simulink model "mf14_100"  (R2023b)
settings: Solver=ode45  StartTime=0.0  StopTime=60  RelTol=1e-4  AbsTol=1e-6
PreLoadFcn:
  | dqesl_f14dat
undefined symbols (not defined in the file): a, b, g, Ka, Kf, Ki, Kq, Md, Mq, Mw, Swg, Ta, Tal, Ts, Uo, Vto, W1, W2, Zd, Zw
libraries: simulink3 x100
(part 1 of 10)
settings Model: Creator=The MathWorks Inc.  LastModifiedBy=dganesan
settings SolverCC: AutoScaleAbsTol=off  AlgebraicLoopSolver=TrustRegion  MaxZcPerStep=1
settings DataIOCC: ExternalInput=[]  InitialState=[]  SaveFormat=Array  SignalLoggingSaveFormat=ModelDataLogs  SaveOutput=off  SaveTime=off  ReturnWorkspaceOutputs=off
settings OptimizationCC: BlockReduction=off  BooleanDataType=off  ExpressionDepthLimit=2147483647  InitFltsAndDblsToZero=on  LifeSpan=inf
settings DebuggingCC: SaveWithParameterizedLinksMsg=none  UnderspecifiedInitializationDetection=Classic  MergeDetectMultiDrivingBlocksExec=none  SignalResolutionControl=TryResolveAllWithWarning  MultiTaskDSMMsg=warning  MultiTaskCondExecSysMsg=none  IntegerOverflowMsg=none  FcnCallInpInsideContextMsg=warning  UnconnectedInputMsg=warning  UnconnectedOutputMsg=warning  UnconnectedLineMsg=warning  StateNameClashWarn=warning  SFUnexpectedBacktrackingDiag=warning  SFNoUnconditionalDefaultTransitionDiag=warning  SFExecutionAtInitializationDiag=none  IntegerSaturationMsg=none  ArithmeticOperatorsInVariantConditions=warning
settings HardwareCC: ProdBitPerPointer=32  ProdBitPerSizeT=32  ProdBitPerPtrDiffT=32  ProdLargestAtomicFloat=None  ProdIntDivRoundTo=Undefined  ProdEndianess=Unspecified  ProdWordSize=32  ProdHWDeviceType=32-bit Generic
settings ModelReferenceCC: EnableRefExpFcnMdlSchedulingChecks=on  PropagateSignalLabelsOutOfModel=off
settings SFSimCC: SimUseLocalCustomCode=off  CustomCodeUndefinedFunction=UseInterfaceOnly
settings RTWCC: RTWUseLocalCustomCode=off  DLArmComputeVersion=19.05
settings CodeAppCC: StateflowObjectComments=on
settings GRTTargetCC: TargetFcnLib=ansi_tfl_tmw.mat  TargetLangStandard=C89/C90 (ANSI)  CombineOutputUpdateFcns=off  GRTInterface=on
settings ConfigComp: CovMetricSettings=dw  CovSaveCumulativeToWorkspaceVar=on  CovSaveSingleToWorkspaceVar=on  CovExternalEMLEnable=off

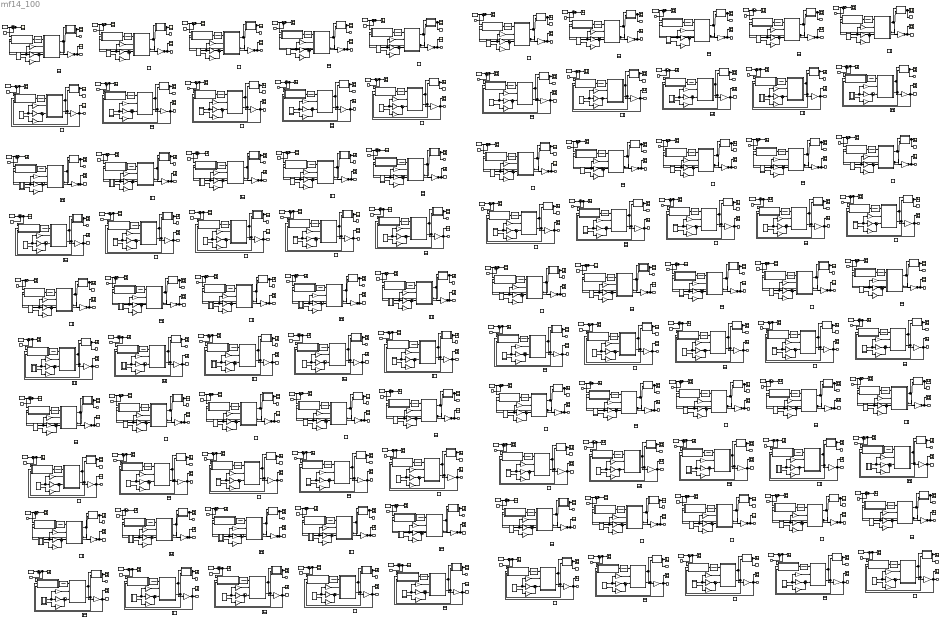
== system mf14_100 ==
  note: F-14 Flight Control
      | (an updated version of this demo is available
      | by running 'sldemo_f14')
  note: Copyright 1990-2010 The MathWorks, Inc.
  note: Copyright 1990-2010 The MathWorks, Inc.
  note: F-14 Flight Control
      | (an updated version of this demo is available
      | by running 'sldemo_f14')
  note: Copyright 1990-2010 The MathWorks, Inc.
  note: F-14 Flight Control
      | (an updated version of this demo is available
      | by running 'sldemo_f14')
  note: Copyright 1990-2010 The MathWorks, Inc.
  note: Copyright 1990-2010 The MathWorks, Inc.
  note: F-14 Flight Control
      | (an updated version of this demo is available
      | by running 'sldemo_f14')
  note: F-14 Flight Control
      | (an updated version of this demo is available
      | by running 'sldemo_f14')
  note: F-14 Flight Control
      | (an updated version of this demo is available
      | by running 'sldemo_f14')
  note: Copyright 1990-2010 The MathWorks, Inc.
  note: Copyright 1990-2010 The MathWorks, Inc.
  note: F-14 Flight Control
      | (an updated version of this demo is available
      | by running 'sldemo_f14')
  note: Copyright 1990-2010 The MathWorks, Inc.
  note: F-14 Flight Control
      | (an updated version of this demo is available
      | by running 'sldemo_f14')
  note: Copyright 1990-2010 The MathWorks, Inc.
  note: F-14 Flight Control
      | (an updated version of this demo is available
      | by running 'sldemo_f14')
  note: Copyright 1990-2010 The MathWorks, Inc.
  note: F-14 Flight Control
      | (an updated version of this demo is available
      | by running 'sldemo_f14')
  note: F-14 Flight Control
      | (an updated version of this demo is available
      | by running 'sldemo_f14')
  note: F-14 Flight Control
      | (an updated version of this demo is available
      | by running 'sldemo_f14')
  note: F-14 Flight Control
      | (an updated version of this demo is available
      | by running 'sldemo_f14')
  note: Copyright 1990-2010 The MathWorks, Inc.
  note: Copyright 1990-2010 The MathWorks, Inc.
  note: F-14 Flight Control
      | (an updated version of this demo is available
      | by running 'sldemo_f14')
  note: Copyright 1990-2010 The MathWorks, Inc.
  note: Copyright 1990-2010 The MathWorks, Inc.
  note: F-14 Flight Control
      | (an updated version of this demo is available
      | by running 'sldemo_f14')
  note: Copyright 1990-2010 The MathWorks, Inc.
  note: F-14 Flight Control
      | (an updated version of this demo is available
      | by running 'sldemo_f14')
  note: Copyright 1990-2010 The MathWorks, Inc.
  note: Copyright 1990-2010 The MathWorks, Inc.
  note: F-14 Flight Control
      | (an updated version of this demo is available
      | by running 'sldemo_f14')
  note: Copyright 1990-2010 The MathWorks, Inc.
  note: F-14 Flight Control
      | (an updated version of this demo is available
      | by running 'sldemo_f14')
  note: Copyright 1990-2010 The MathWorks, Inc.
  note: F-14 Flight Control
      | (an updated version of this demo is available
      | by running 'sldemo_f14')
  note: Copyright 1990-2010 The MathWorks, Inc.
  note: F-14 Flight Control
      | (an updated version of this demo is available
      | by running 'sldemo_f14')
  note: F-14 Flight Control
      | (an updated version of this demo is available
      | by running 'sldemo_f14')
  note: F-14 Flight Control
      | (an updated version of this demo is available
      | by running 'sldemo_f14')
  note: F-14 Flight Control
      | (an updated version of this demo is available
      | by running 'sldemo_f14')
  note: Copyright 1990-2010 The MathWorks, Inc.
  note: Copyright 1990-2010 The MathWorks, Inc.
  note: F-14 Flight Control
      | (an updated version of this demo is available
      | by running 'sldemo_f14')
  note: Copyright 1990-2010 The MathWorks, Inc.
  note: Copyright 1990-2010 The MathWorks, Inc.
  note: F-14 Flight Control
      | (an updated version of this demo is available
      | by running 'sldemo_f14')
  note: Copyright 1990-2010 The MathWorks, Inc.
  note: F-14 Flight Control
      | (an updated version of this demo is available
      | by running 'sldemo_f14')
  note: Copyright 1990-2010 The MathWorks, Inc.
  note: Copyright 1990-2010 The MathWorks, Inc.
  note: F-14 Flight Control
      | (an updated version of this demo is available
      | by running 'sldemo_f14')
  note: Copyright 1990-2010 The MathWorks, Inc.
  note: F-14 Flight Control
      | (an updated version of this demo is available
      | by running 'sldemo_f14')
  note: Copyright 1990-2010 The MathWorks, Inc.
  note: F-14 Flight Control
      | (an updated version of this demo is available
      | by running 'sldemo_f14')
  note: Copyright 1990-2010 The MathWorks, Inc.
  note: F-14 Flight Control
      | (an updated version of this demo is available
      | by running 'sldemo_f14')
  note: F-14 Flight Control
      | (an updated version of this demo is available
      | by running 'sldemo_f14')
  note: F-14 Flight Control
      | (an updated version of this demo is available
      | by running 'sldemo_f14')
  note: F-14 Flight Control
      | (an updated version of this demo is available
      | by running 'sldemo_f14')
  note: Copyright 1990-2010 The MathWorks, Inc.
  note: Copyright 1990-2010 The MathWorks, Inc.
  note: F-14 Flight Control
      | (an updated version of this demo is available
      | by running 'sldemo_f14')
  note: Copyright 1990-2010 The MathWorks, Inc.
  note: Copyright 1990-2010 The MathWorks, Inc.
  note: F-14 Flight Control
      | (an updated version of this demo is available
      | by running 'sldemo_f14')
  note: Copyright 1990-2010 The MathWorks, Inc.
  note: F-14 Flight Control
      | (an updated version of this demo is available
      | by running 'sldemo_f14')
  note: Copyright 1990-2010 The MathWorks, Inc.
  note: Copyright 1990-2010 The MathWorks, Inc.
  note: F-14 Flight Control
      | (an updated version of this demo is available
      | by running 'sldemo_f14')
  note: Copyright 1990-2010 The MathWorks, Inc.
  note: F-14 Flight Control
      | (an updated version of this demo is available
      | by running 'sldemo_f14')
  note: Copyright 1990-2010 The MathWorks, Inc.
  note: F-14 Flight Control
      | (an updated version of this demo is available
      | by running 'sldemo_f14')
  note: Copyright 1990-2010 The MathWorks, Inc.
  note: F-14 Flight Control
      | (an updated version of this demo is available
      | by running 'sldemo_f14')
  note: F-14 Flight Control
      | (an updated version of this demo is available
      | by running 'sldemo_f14')
  note: F-14 Flight Control
      | (an updated version of this demo is available
      | by running 'sldemo_f14')
  note: F-14 Flight Control
      | (an updated version of this demo is available
      | by running 'sldemo_f14')
  note: Copyright 1990-2010 The MathWorks, Inc.
  note: Copyright 1990-2010 The MathWorks, Inc.
  note: F-14 Flight Control
      | (an updated version of this demo is available
      | by running 'sldemo_f14')
  note: Copyright 1990-2010 The MathWorks, Inc.
  note: Copyright 1990-2010 The MathWorks, Inc.
  note: F-14 Flight Control
      | (an updated version of this demo is available
      | by running 'sldemo_f14')
  note: Copyright 1990-2010 The MathWorks, Inc.
  note: F-14 Flight Control
      | (an updated version of this demo is available
      | by running 'sldemo_f14')
  note: Copyright 1990-2010 The MathWorks, Inc.
  note: Copyright 1990-2010 The MathWorks, Inc.
  note: F-14 Flight Control
      | (an updated version of this demo is available
      | by running 'sldemo_f14')
  note: Copyright 1990-2010 The MathWorks, Inc.
  note: F-14 Flight Control
      | (an updated version of this demo is available
      | by running 'sldemo_f14')
  note: Copyright 1990-2010 The MathWorks, Inc.
  note: F-14 Flight Control
      | (an updated version of this demo is available
      | by running 'sldemo_f14')
  note: Copyright 1990-2010 The MathWorks, Inc.
  note: F-14 Flight Control
      | (an updated version of this demo is available
      | by running 'sldemo_f14')
  note: F-14 Flight Control
      | (an updated version of this demo is available
      | by running 'sldemo_f14')
  note: Copyright 1990-2010 The MathWorks, Inc.
  note: F-14 Flight Control
      | (an updated version of this demo is available
      | by running 'sldemo_f14')
  note: F-14 Flight Control
      | (an updated version of this demo is available
      | by running 'sldemo_f14')
  note: F-14 Flight Control
      | (an updated version of this demo is available
      | by running 'sldemo_f14')
  note: Copyright 1990-2010 The MathWorks, Inc.
  note: Copyright 1990-2010 The MathWorks, Inc.
  note: Copyright 1990-2010 The MathWorks, Inc.
  note: Copyright 1990-2010 The MathWorks, Inc.
  note: Copyright 1990-2010 The MathWorks, Inc.
  note: F-14 Flight Control
      | (an updated version of this demo is available
      | by running 'sldemo_f14')
  note: Copyright 1990-2010 The MathWorks, Inc.
  note: Copyright 1990-2010 The MathWorks, Inc.
  note: F-14 Flight Control
      | (an updated version of this demo is available
      | by running 'sldemo_f14')
  note: F-14 Flight Control
      | (an updated version of this demo is available
      | by running 'sldemo_f14')
  note: F-14 Flight Control
      | (an updated version of this demo is available
      | by running 'sldemo_f14')
  note: F-14 Flight Control
      | (an updated version of this demo is available
      | by running 'sldemo_f14')
  note: F-14 Flight Control
      | (an updated version of this demo is available
      | by running 'sldemo_f14')
  note: Copyright 1990-2010 The MathWorks, Inc.
  note: Copyright 1990-2010 The MathWorks, Inc.
  note: F-14 Flight Control
      | (an updated version of this demo is available
      | by running 'sldemo_f14')
  note: Copyright 1990-2010 The MathWorks, Inc.
  note: Copyright 1990-2010 The MathWorks, Inc.
  note: F-14 Flight Control
      | (an updated version of this demo is available
      | by running 'sldemo_f14')
  note: F-14 Flight Control
      | (an updated version of this demo is available
      | by running 'sldemo_f14')
  note: Copyright 1990-2010 The MathWorks, Inc.
  note: F-14 Flight Control
      | (an updated version of this demo is available
      | by running 'sldemo_f14')
  note: Copyright 1990-2010 The MathWorks, Inc.
  note: F-14 Flight Control
      | (an updated version of this demo is available
      | by running 'sldemo_f14')
  note: F-14 Flight Control
      | (an updated version of this demo is available
      | by running 'sldemo_f14')
  note: Copyright 1990-2010 The MathWorks, Inc.
  note: F-14 Flight Control
      | (an updated version of this demo is available
      | by running 'sldemo_f14')
  note: F-14 Flight Control
      | (an updated version of this demo is available
      | by running 'sldemo_f14')
  note: F-14 Flight Control
      | (an updated version of this demo is available
      | by running 'sldemo_f14')
  note: Copyright 1990-2010 The MathWorks, Inc.
  note: Copyright 1990-2010 The MathWorks, Inc.
  note: F-14 Flight Control
      | (an updated version of this demo is available
      | by running 'sldemo_f14')
  note: F-14 Flight Control
      | (an updated version of this demo is available
      | by running 'sldemo_f14')
  note: F-14 Flight Control
      | (an updated version of this demo is available
      | by running 'sldemo_f14')
  note: F-14 Flight Control
      | (an updated version of this demo is available
      | by running 'sldemo_f14')
  note: Copyright 1990-2010 The MathWorks, Inc.
  note: F-14 Flight Control
      | (an updated version of this demo is available
      | by running 'sldemo_f14')
  note: Copyright 1990-2010 The MathWorks, Inc.
  note: Copyright 1990-2010 The MathWorks, Inc.
  note: F-14 Flight Control
      | (an updated version of this demo is available
      | by running 'sldemo_f14')
  note: Copyright 1990-2010 The MathWorks, Inc.
  note: Copyright 1990-2010 The MathWorks, Inc.
  note: Copyright 1990-2010 The MathWorks, Inc.
  note: F-14 Flight Control
      | (an updated version of this demo is available
      | by running 'sldemo_f14')
  note: Copyright 1990-2010 The MathWorks, Inc.
  note: Copyright 1990-2010 The MathWorks, Inc.
  note: Copyright 1990-2010 The MathWorks, Inc.
  note: F-14 Flight Control
      | (an updated version of this demo is available
      | by running 'sldemo_f14')
  note: F-14 Flight Control
      | (an updated version of this demo is available
      | by running 'sldemo_f14')
  note: Copyright 1990-2010 The MathWorks, Inc.
  note: F-14 Flight Control
      | (an updated version of this demo is available
      | by running 'sldemo_f14')
  note: Copyright 1990-2010 The MathWorks, Inc.
  note: Copyright 1990-2010 The MathWorks, Inc.
  note: F-14 Flight Control
      | (an updated version of this demo is available
      | by running 'sldemo_f14')
  note: Copyright 1990-2010 The MathWorks, Inc.
  note: Copyright 1990-2010 The MathWorks, Inc.
  note: Copyright 1990-2010 The MathWorks, Inc.
  note: F-14 Flight Control
      | (an updated version of this demo is available
      | by running 'sldemo_f14')
  note: F-14 Flight Control
      | (an updated version of this demo is available
      | by running 'sldemo_f14')
  note: Copyright 1990-2010 The MathWorks, Inc.
  note: Copyright 1990-2010 The MathWorks, Inc.
  note: Copyright 1990-2010 The MathWorks, Inc.
  note: F-14 Flight Control
      | (an updated version of this demo is available
      | by running 'sldemo_f14')
  note: Copyright 1990-2010 The MathWorks, Inc.
  note: F-14 Flight Control
      | (an updated version of this demo is available
      | by running 'sldemo_f14')
  note: F-14 Flight Control
      | (an updated version of this demo is available
      | by running 'sldemo_f14')
  note: Copyright 1990-2010 The MathWorks, Inc.
  note: Copyright 1990-2010 The MathWorks, Inc.
  note: Copyright 1990-2010 The MathWorks, Inc.
  note: F-14 Flight Control
      | (an updated version of this demo is available
      | by running 'sldemo_f14')
  note: Copyright 1990-2010 The MathWorks, Inc.
  note: Copyright 1990-2010 The MathWorks, Inc.
  note: F-14 Flight Control
      | (an updated version of this demo is available
      | by running 'sldemo_f14')
  note: F-14 Flight Control
      | (an updated version of this demo is available
      | by running 'sldemo_f14')
  note: F-14 Flight Control
      | (an updated version of this demo is available
      | by running 'sldemo_f14')
  note: F-14 Flight Control
      | (an updated version of this demo is available
      | by running 'sldemo_f14')
  note: F-14 Flight Control
      | (an updated version of this demo is available
      | by running 'sldemo_f14')
  note: F-14 Flight Control
      | (an updated version of this demo is available
      | by running 'sldemo_f14')
  note: Copyright 1990-2010 The MathWorks, Inc.
  note: Copyright 1990-2010 The MathWorks, Inc.
  note: Copyright 1990-2010 The MathWorks, Inc.
  note: F-14 Flight Control
      | (an updated version of this demo is available
      | by running 'sldemo_f14')
  note: Copyright 1990-2010 The MathWorks, Inc.
  note: Copyright 1990-2010 The MathWorks, Inc.
  note: F-14 Flight Control
      | (an updated version of this demo is available
      | by running 'sldemo_f14')
  note: F-14 Flight Control
      | (an updated version of this demo is available
      | by running 'sldemo_f14')
  note: F-14 Flight Control
      | (an updated version of this demo is available
      | by running 'sldemo_f14')
  note: F-14 Flight Control
      | (an updated version of this demo is available
      | by running 'sldemo_f14')
  note: Copyright 1990-2010 The MathWorks, Inc.
  note: F-14 Flight Control
      | (an updated version of this demo is available
      | by running 'sldemo_f14')
  note: F-14 Flight Control
      | (an updated version of this demo is available
      | by running 'sldemo_f14')
  note: F-14 Flight Control
      | (an updated version of this demo is available
      | by running 'sldemo_f14')
  note: Copyright 1990-2010 The MathWorks, Inc.
  note: Copyright 1990-2010 The MathWorks, Inc.
  note: Copyright 1990-2010 The MathWorks, Inc.
  u : Inport
  u1 : Inport  Port=2
  u2 : Inport  Port=3
  u3 : Inport  Port=4
  u4 : Inport  Port=5
  u5 : Inport  Port=6
  u6 : Inport  Port=7
  u7 : Inport  Port=8
  u8 : Inport  Port=9
  u9 : Inport  Port=10
  u10 : Inport  Port=11
  u11 : Inport  Port=12
  u12 : Inport  Port=13
  u13 : Inport  Port=14
  u14 : Inport  Port=15
  u15 : Inport  Port=16
  u16 : Inport  Port=17
  u17 : Inport  Port=18
  u18 : Inport  Port=19
  u19 : Inport  Port=20
  u20 : Inport  Port=21
  u21 : Inport  Port=22
  u22 : Inport  Port=23
  u23 : Inport  Port=24
  u24 : Inport  Port=25
  u25 : Inport  Port=26
  u26 : Inport  Port=27
  u27 : Inport  Port=28
  u28 : Inport  Port=29
  u29 : Inport  Port=30
  u30 : Inport  Port=31
  u31 : Inport  Port=32
  u32 : Inport  Port=33
  u33 : Inport  Port=34
  u34 : Inport  Port=35
  u35 : Inport  Port=36
  u36 : Inport  Port=37
  u37 : Inport  Port=38
  u38 : Inport  Port=39
  u39 : Inport  Port=40
  u40 : Inport  Port=41
  u41 : Inport  Port=42
  u42 : Inport  Port=43
  u43 : Inport  Port=44
  u44 : Inport  Port=45
  u45 : Inport  Port=46
  u46 : Inport  Port=47
  u47 : Inport  Port=48
  u48 : Inport  Port=49
  u49 : Inport  Port=50
  u50 : Inport  Port=51
  u51 : Inport  Port=52
  u52 : Inport  Port=53
  u53 : Inport  Port=54
  u54 : Inport  Port=55
  u55 : Inport  Port=56
  u56 : Inport  Port=57
  u57 : Inport  Port=58
  u58 : Inport  Port=59
  u59 : Inport  Port=60
  u60 : Inport  Port=61
  u61 : Inport  Port=62
  u62 : Inport  Port=63
  u63 : Inport  Port=64
  u64 : Inport  Port=65
  u65 : Inport  Port=66
  u66 : Inport  Port=67
  u67 : Inport  Port=68
  u68 : Inport  Port=69
  u69 : Inport  Port=70
  u70 : Inport  Port=71
  u71 : Inport  Port=72
  u72 : Inport  Port=73
  u73 : Inport  Port=74
  u74 : Inport  Port=75
  u75 : Inport  Port=76
  u76 : Inport  Port=77
  u77 : Inport  Port=78
  u78 : Inport  Port=79
  u79 : Inport  Port=80
  u80 : Inport  Port=81
  u81 : Inport  Port=82
  u82 : Inport  Port=83
  u83 : Inport  Port=84
  u84 : Inport  Port=85
  u85 : Inport  Port=86
  u86 : Inport  Port=87
  u87 : Inport  Port=88
  u88 : Inport  Port=89
  u89 : Inport  Port=90
  u90 : Inport  Port=91
  u91 : Inport  Port=92
  u92 : Inport  Port=93
  u93 : Inport  Port=94
  u94 : Inport  Port=95
  u95 : Inport  Port=96
  u96 : Inport  Port=97
  u97 : Inport  Port=98
  u98 : Inport  Port=99
  u99 : Inport  Port=100
  Actuator Model{,1..99} (100 alike) : TransferFcn  Denominator=[ Ta, 1]
  Aircraft Dynamics Model : Subsystem
  Aircraft Dynamics Model1 : Subsystem
  Aircraft Dynamics Model10 : Subsystem
  Aircraft Dynamics Model11 : Subsystem
  Aircraft Dynamics Model12 : Subsystem
  Aircraft Dynamics Model13 : Subsystem
  Aircraft Dynamics Model14 : Subsystem
  Aircraft Dynamics Model15 : Subsystem
  Aircraft Dynamics Model16 : Subsystem
  Aircraft Dynamics Model17 : Subsystem
  Aircraft Dynamics Model18 : Subsystem
  Aircraft Dynamics Model19 : Subsystem
  Aircraft Dynamics Model2 : Subsystem
  Aircraft Dynamics Model20 : Subsystem
  Aircraft Dynamics Model21 : Subsystem
  Aircraft Dynamics Model22 : Subsystem
  Aircraft Dynamics Model23 : Subsystem
  Aircraft Dynamics Model24 : Subsystem
  Aircraft Dynamics Model25 : Subsystem
  Aircraft Dynamics Model26 : Subsystem
  Aircraft Dynamics Model27 : Subsystem
  Aircraft Dynamics Model28 : Subsystem
  Aircraft Dynamics Model29 : Subsystem
  Aircraft Dynamics Model3 : Subsystem
  Aircraft Dynamics Model30 : Subsystem
  Aircraft Dynamics Model31 : Subsystem
  Aircraft Dynamics Model32 : Subsystem
  Aircraft Dynamics Model33 : Subsystem
  Aircraft Dynamics Model34 : Subsystem
  Aircraft Dynamics Model35 : Subsystem
  Aircraft Dynamics Model36 : Subsystem
  Aircraft Dynamics Model37 : Subsystem
  Aircraft Dynamics Model38 : Subsystem
  Aircraft Dynamics Model39 : Subsystem
  Aircraft Dynamics Model4 : Subsystem
  Aircraft Dynamics Model40 : Subsystem
  Aircraft Dynamics Model41 : Subsystem
  Aircraft Dynamics Model42 : Subsystem
  Aircraft Dynamics Model43 : Subsystem
  Aircraft Dynamics Model44 : Subsystem
  Aircraft Dynamics Model45 : Subsystem
  Aircraft Dynamics Model46 : Subsystem
  Aircraft Dynamics Model47 : Subsystem
  Aircraft Dynamics Model48 : Subsystem
  Aircraft Dynamics Model49 : Subsystem
  Aircraft Dynamics Model5 : Subsystem
  Aircraft Dynamics Model50 : Subsystem
  Aircraft Dynamics Model51 : Subsystem
  Aircraft Dynamics Model52 : Subsystem
  Aircraft Dynamics Model53 : Subsystem
  Aircraft Dynamics Model54 : Subsystem
  Aircraft Dynamics Model55 : Subsystem
  Aircraft Dynamics Model56 : Subsystem
  Aircraft Dynamics Model57 : Subsystem
  Aircraft Dynamics Model58 : Subsystem
  Aircraft Dynamics Model59 : Subsystem
  Aircraft Dynamics Model6 : Subsystem
  Aircraft Dynamics Model60 : Subsystem
  Aircraft Dynamics Model61 : Subsystem
  Aircraft Dynamics Model62 : Subsystem
  Aircraft Dynamics Model63 : Subsystem
  Aircraft Dynamics Model64 : Subsystem
  Aircraft Dynamics Model65 : Subsystem
  Aircraft Dynamics Model66 : Subsystem
  Aircraft Dynamics Model67 : Subsystem
  Aircraft Dynamics Model68 : Subsystem
  Aircraft Dynamics Model69 : Subsystem
  Aircraft Dynamics Model7 : Subsystem
  Aircraft Dynamics Model70 : Subsystem
  Aircraft Dynamics Model71 : Subsystem
  Aircraft Dynamics Model72 : Subsystem
  Aircraft Dynamics Model73 : Subsystem
  Aircraft Dynamics Model74 : Subsystem
  Aircraft Dynamics Model75 : Subsystem
  Aircraft Dynamics Model76 : Subsystem
  Aircraft Dynamics Model77 : Subsystem
  Aircraft Dynamics Model78 : Subsystem
  Aircraft Dynamics Model79 : Subsystem
  Aircraft Dynamics Model8 : Subsystem
  Aircraft Dynamics Model80 : Subsystem
  Aircraft Dynamics Model81 : Subsystem
  Aircraft Dynamics Model82 : Subsystem
  Aircraft Dynamics Model83 : Subsystem
  Aircraft Dynamics Model84 : Subsystem
  Aircraft Dynamics Model85 : Subsystem
  Aircraft Dynamics Model86 : Subsystem
  Aircraft Dynamics Model87 : Subsystem
  Aircraft Dynamics Model88 : Subsystem
  Aircraft Dynamics Model89 : Subsystem
  Aircraft Dynamics Model9 : Subsystem
  Aircraft Dynamics Model90 : Subsystem
  Aircraft Dynamics Model91 : Subsystem
  Aircraft Dynamics Model92 : Subsystem
  Aircraft Dynamics Model93 : Subsystem
  Aircraft Dynamics Model94 : Subsystem
  Aircraft Dynamics Model95 : Subsystem
  Aircraft Dynamics Model96 : Subsystem
  Aircraft Dynamics Model97 : Subsystem
  Aircraft Dynamics Model98 : Subsystem
  Aircraft Dynamics Model99 : Subsystem
  Angle of Attack{,1..99} (100 alike) : Scope
  Controller : Subsystem
  Controller1 : Subsystem
  Controller10 : Subsystem
  Controller11 : Subsystem
  Controller12 : Subsystem
  Controller13 : Subsystem
  Controller14 : Subsystem
  Controller15 : Subsystem
  Controller16 : Subsystem
  Controller17 : Subsystem
  Controller18 : Subsystem
  Controller19 : Subsystem
  Controller2 : Subsystem
  Controller20 : Subsystem
  Controller21 : Subsystem
  Controller22 : Subsystem
  Controller23 : Subsystem
  Controller24 : Subsystem
  Controller25 : Subsystem
  Controller26 : Subsystem
  Controller27 : Subsystem
  Controller28 : Subsystem
  Controller29 : Subsystem
  Controller3 : Subsystem
  Controller30 : Subsystem
  Controller31 : Subsystem
  Controller32 : Subsystem
  Controller33 : Subsystem
  Controller34 : Subsystem
  Controller35 : Subsystem
  Controller36 : Subsystem
  Controller37 : Subsystem
  Controller38 : Subsystem
  Controller39 : Subsystem
  Controller4 : Subsystem
  Controller40 : Subsystem
  Controller41 : Subsystem
  Controller42 : Subsystem
  Controller43 : Subsystem
  Controller44 : Subsystem
  Controller45 : Subsystem
  Controller46 : Subsystem
  Controller47 : Subsystem
  Controller48 : Subsystem
  Controller49 : Subsystem
  Controller5 : Subsystem
  Controller50 : Subsystem
  Controller51 : Subsystem
  Controller52 : Subsystem
  Controller53 : Subsystem
  Controller54 : Subsystem
  Controller55 : Subsystem
  Controller56 : Subsystem
  Controller57 : Subsystem
  Controller58 : Subsystem
  Controller59 : Subsystem
  Controller6 : Subsystem
  Controller60 : Subsystem
  Controller61 : Subsystem
  Controller62 : Subsystem
  Controller63 : Subsystem
  Controller64 : Subsystem
  Controller65 : Subsystem
  Controller66 : Subsystem
  Controller67 : Subsystem
  Controller68 : Subsystem
  Controller69 : Subsystem
  Controller7 : Subsystem
  Controller70 : Subsystem
  Controller71 : Subsystem
  Controller72 : Subsystem
  Controller73 : Subsystem
  Controller74 : Subsystem
  Controller75 : Subsystem
  Controller76 : Subsystem
  Controller77 : Subsystem
  Controller78 : Subsystem
  Controller79 : Subsystem
  Controller8 : Subsystem
  Controller80 : Subsystem
  Controller81 : Subsystem
  Controller82 : Subsystem
  Controller83 : Subsystem
  Controller84 : Subsystem
  Controller85 : Subsystem
  Controller86 : Subsystem
  Controller87 : Subsystem
  Controller88 : Subsystem
  Controller89 : Subsystem
  Controller9 : Subsystem
  Controller90 : Subsystem
  Controller91 : Subsystem
  Controller92 : Subsystem
  Controller93 : Subsystem
  Controller94 : Subsystem
  Controller95 : Subsystem
  Controller96 : Subsystem
  Controller97 : Subsystem
  Controller98 : Subsystem
  Controller99 : Subsystem
  Dryden Wind Gust Models : Subsystem
  Dryden Wind Gust Models1 : Subsystem
  Dryden Wind Gust Models10 : Subsystem
  Dryden Wind Gust Models11 : Subsystem
  Dryden Wind Gust Models12 : Subsystem
  Dryden Wind Gust Models13 : Subsystem
  Dryden Wind Gust Models14 : Subsystem
  Dryden Wind Gust Models15 : Subsystem
  Dryden Wind Gust Models16 : Subsystem
  Dryden Wind Gust Models17 : Subsystem
  Dryden Wind Gust Models18 : Subsystem
  Dryden Wind Gust Models19 : Subsystem
  Dryden Wind Gust Models2 : Subsystem
  Dryden Wind Gust Models20 : Subsystem
  Dryden Wind Gust Models21 : Subsystem
  Dryden Wind Gust Models22 : Subsystem
  Dryden Wind Gust Models23 : Subsystem
  Dryden Wind Gust Models24 : Subsystem
  Dryden Wind Gust Models25 : Subsystem
  Dryden Wind Gust Models26 : Subsystem
  Dryden Wind Gust Models27 : Subsystem
  Dryden Wind Gust Models28 : Subsystem
  Dryden Wind Gust Models29 : Subsystem
  Dryden Wind Gust Models3 : Subsystem
  Dryden Wind Gust Models30 : Subsystem
  Dryden Wind Gust Models31 : Subsystem
  Dryden Wind Gust Models32 : Subsystem
  Dryden Wind Gust Models33 : Subsystem
  Dryden Wind Gust Models34 : Subsystem
  Dryden Wind Gust Models35 : Subsystem
  Dryden Wind Gust Models36 : Subsystem
  Dryden Wind Gust Models37 : Subsystem
  Dryden Wind Gust Models38 : Subsystem
  Dryden Wind Gust Models39 : Subsystem
  Dryden Wind Gust Models4 : Subsystem
  Dryden Wind Gust Models40 : Subsystem
  Dryden Wind Gust Models41 : Subsystem
  Dryden Wind Gust Models42 : Subsystem
  Dryden Wind Gust Models43 : Subsystem
  Dryden Wind Gust Models44 : Subsystem
  Dryden Wind Gust Models45 : Subsystem
  Dryden Wind Gust Models46 : Subsystem
  Dryden Wind Gust Models47 : Subsystem
  Dryden Wind Gust Models48 : Subsystem
  Dryden Wind Gust Models49 : Subsystem
  Dryden Wind Gust Models5 : Subsystem
  Dryden Wind Gust Models50 : Subsystem
  Dryden Wind Gust Models51 : Subsystem
  Dryden Wind Gust Models52 : Subsystem
  Dryden Wind Gust Models53 : Subsystem
  Dryden Wind Gust Models54 : Subsystem
  Dryden Wind Gust Models55 : Subsystem
  Dryden Wind Gust Models56 : Subsystem
  Dryden Wind Gust Models57 : Subsystem
  Dryden Wind Gust Models58 : Subsystem
  Dryden Wind Gust Models59 : Subsystem
  Dryden Wind Gust Models6 : Subsystem
  Dryden Wind Gust Models60 : Subsystem
  Dryden Wind Gust Models61 : Subsystem
  Dryden Wind Gust Models62 : Subsystem
  Dryden Wind Gust Models63 : Subsystem
  Dryden Wind Gust Models64 : Subsystem
  Dryden Wind Gust Models65 : Subsystem
  Dryden Wind Gust Models66 : Subsystem
  Dryden Wind Gust Models67 : Subsystem
  Dryden Wind Gust Models68 : Subsystem
  Dryden Wind Gust Models69 : Subsystem
  Dryden Wind Gust Models7 : Subsystem
  Dryden Wind Gust Models70 : Subsystem
  Dryden Wind Gust Models71 : Subsystem
  Dryden Wind Gust Models72 : Subsystem
  Dryden Wind Gust Models73 : Subsystem
  Dryden Wind Gust Models74 : Subsystem
  Dryden Wind Gust Models75 : Subsystem
  Dryden Wind Gust Models76 : Subsystem
  Dryden Wind Gust Models77 : Subsystem
  Dryden Wind Gust Models78 : Subsystem
  Dryden Wind Gust Models79 : Subsystem
  Dryden Wind Gust Models8 : Subsystem
  Dryden Wind Gust Models80 : Subsystem
  Dryden Wind Gust Models81 : Subsystem
  Dryden Wind Gust Models82 : Subsystem
  Dryden Wind Gust Models83 : Subsystem
  Dryden Wind Gust Models84 : Subsystem
  Dryden Wind Gust Models85 : Subsystem
  Dryden Wind Gust Models86 : Subsystem
  Dryden Wind Gust Models87 : Subsystem
  Dryden Wind Gust Models88 : Subsystem
  Dryden Wind Gust Models89 : Subsystem
  Dryden Wind Gust Models9 : Subsystem
  Dryden Wind Gust Models90 : Subsystem
  Dryden Wind Gust Models91 : Subsystem
  Dryden Wind Gust Models92 : Subsystem
  Dryden Wind Gust Models93 : Subsystem
  Dryden Wind Gust Models94 : Subsystem
  Dryden Wind Gust Models95 : Subsystem
  Dryden Wind Gust Models96 : Subsystem
  Dryden Wind Gust Models97 : Subsystem
  Dryden Wind Gust Models98 : Subsystem
  Dryden Wind Gust Models99 : Subsystem
  Gain{,3,8,12,15,20,24,27,33,38,40,44,47,53,57,60,63,67,72,78,80,84,87,93,97,100,103,107,112,118,120,124,127,133,137,140,143,147,152,158,160,164,167,173,177,180,183,187,192,198,200,203,206,210,216,222,224..225,229,232,239,243,247,250,254,257,260,266,269,273,276,283,287,291,294,298,304,310,313,317,320,323,327,332,335,339,342,349,353,357,360,364,370,376,378..379,383,386,393,397} (100 alike) : Gain  Gain=Zw  SaturateOnIntegerOverflow=on  OutDataTypeStr=Inherit: Same as input  ParamDataTypeStr=Inherit: Same as input
  Gain{1,4,9,13,16,21,25,28,34,39,41,45,48,54,58,61,68,73..74,79,81,85,88,94,98,101,108,113..114,119,121,125,128,134,138,141,148,153..154,159,161,165,168,174,178,181,188,193..194,199,201,204,211,217..218,223,226,230,233,235,240,244,248,255,261..262,267..268,270,274,277,284,288,292,299,305..306,311,314,318,321,328,333..334,336,340,343,350,354,358,365,371..372,377,380,384,387,389,394,398} (100 alike) : Gain  Gain=Mq  SaturateOnIntegerOverflow=on  OutDataTypeStr=Inherit: Same as input  ParamDataTypeStr=Inherit: Same as input
  Gain{2,6,10,14,18,22,26,30,32,36,42,46,50,52,55,59,64,66,70,76,82,86,90,92,95,99,104,106,110,116,122,126,130,132,135,139,144,146,150,156,162,166,170,172,175,179,184,186,190,196,202,207,209,214,220,227,231,236,238,241,245..246,251,253,258,264,271,275,280,282,285,289..290,295,297,302,308,312,315,319,324,326,330,337,341,346,348,351,355..356,361,363,368,374,381,385,390,392,395,399} (100 alike) : Gain  Gain=Mw  SaturateOnIntegerOverflow=on  OutDataTypeStr=Inherit: Same as input  ParamDataTypeStr=Inherit: Same as input
  Gain{5,7,11,17,19,23,29,31,35,37,43,49,51,56,62,65,69,71,75,77,83,89,91,96,102,105,109,111,115,117,123,129,131,136,142,145,149,151,155,157,163,169,171,176,182,185,189,191,195,197,205,208,212..213,215,219,221,228,234,237,242,249,252,256,259,263,265,272,278..279,281,286,293,296,300..301,303,307,309,316,322,325,329,331,338,344..345,347,352,359,362,366..367,369,373,375,382,388,391,396} (100 alike) : Gain  Gain=1/Uo  SaturateOnIntegerOverflow=on  OutDataTypeStr=Inherit: Same as input  ParamDataTypeStr=Inherit: Same as input
  More Info1 : Subsystem
      settings: OpenFcn=showdemo('sldemo_f14')
      mask Display: disp('?')
  More Info10 : Subsystem
      settings: OpenFcn=showdemo('sldemo_f14')
      mask Display: disp('?')
  More Info100 : Subsystem
      settings: OpenFcn=showdemo('sldemo_f14')
      mask Display: disp('?')
  More Info11 : Subsystem
      settings: OpenFcn=showdemo('sldemo_f14')
      mask Display: disp('?')
  More Info12 : Subsystem
      settings: OpenFcn=showdemo('sldemo_f14')
      mask Display: disp('?')
  More Info13 : Subsystem
      settings: OpenFcn=showdemo('sldemo_f14')
      mask Display: disp('?')
  More Info14 : Subsystem
      settings: OpenFcn=showdemo('sldemo_f14')
      mask Display: disp('?')
  More Info15 : Subsystem
      settings: OpenFcn=showdemo('sldemo_f14')
      mask Display: disp('?')
  More Info16 : Subsystem
      settings: OpenFcn=showdemo('sldemo_f14')
      mask Display: disp('?')
  More Info17 : Subsystem
      settings: OpenFcn=showdemo('sldemo_f14')
      mask Display: disp('?')
  More Info18 : Subsystem
      settings: OpenFcn=showdemo('sldemo_f14')
      mask Display: disp('?')
  More Info19 : Subsystem
      settings: OpenFcn=showdemo('sldemo_f14')
      mask Display: disp('?')
  More Info2 : Subsystem
      settings: OpenFcn=showdemo('sldemo_f14')
      mask Display: disp('?')
  More Info20 : Subsystem
      settings: OpenFcn=showdemo('sldemo_f14')
      mask Display: disp('?')
  More Info21 : Subsystem
      settings: OpenFcn=showdemo('sldemo_f14')
      mask Display: disp('?')
  More Info22 : Subsystem
      settings: OpenFcn=showdemo('sldemo_f14')
      mask Display: disp('?')
  More Info23 : Subsystem
      settings: OpenFcn=showdemo('sldemo_f14')
      mask Display: disp('?')
  More Info24 : Subsystem
      settings: OpenFcn=showdemo('sldemo_f14')
      mask Display: disp('?')
  More Info25 : Subsystem
      settings: OpenFcn=showdemo('sldemo_f14')
      mask Display: disp('?')
  More Info26 : Subsystem
      settings: OpenFcn=showdemo('sldemo_f14')
      mask Display: disp('?')
  More Info27 : Subsystem
      settings: OpenFcn=showdemo('sldemo_f14')
      mask Display: disp('?')
  More Info28 : Subsystem
      settings: OpenFcn=showdemo('sldemo_f14')
      mask Display: disp('?')
  More Info29 : Subsystem
      settings: OpenFcn=showdemo('sldemo_f14')
      mask Display: disp('?')
  More Info3 : Subsystem
      settings: OpenFcn=showdemo('sldemo_f14')
      mask Display: disp('?')
  More Info30 : Subsystem
      settings: OpenFcn=showdemo('sldemo_f14')
      mask Display: disp('?')
  More Info31 : Subsystem
      settings: OpenFcn=showdemo('sldemo_f14')
      mask Display: disp('?')
  More Info32 : Subsystem
      settings: OpenFcn=showdemo('sldemo_f14')
      mask Display: disp('?')
  More Info33 : Subsystem
      settings: OpenFcn=showdemo('sldemo_f14')
      mask Display: disp('?')
  More Info34 : Subsystem
      settings: OpenFcn=showdemo('sldemo_f14')
      mask Display: disp('?')
  More Info35 : Subsystem
      settings: OpenFcn=showdemo('sldemo_f14')
      mask Display: disp('?')
  More Info36 : Subsystem
      settings: OpenFcn=showdemo('sldemo_f14')
      mask Display: disp('?')
  More Info37 : Subsystem
      settings: OpenFcn=showdemo('sldemo_f14')
      mask Display: disp('?')
  More Info38 : Subsystem
      settings: OpenFcn=showdemo('sldemo_f14')
      mask Display: disp('?')
  More Info39 : Subsystem
      settings: OpenFcn=showdemo('sldemo_f14')
      mask Display: disp('?')
  More Info4 : Subsystem
      settings: OpenFcn=showdemo('sldemo_f14')
      mask Display: disp('?')
  More Info40 : Subsystem
      settings: OpenFcn=showdemo('sldemo_f14')
      mask Display: disp('?')
  More Info41 : Subsystem
      settings: OpenFcn=showdemo('sldemo_f14')
      mask Display: disp('?')
  More Info42 : Subsystem
      settings: OpenFcn=showdemo('sldemo_f14')
      mask Display: disp('?')
  More Info43 : Subsystem
      settings: OpenFcn=showdemo('sldemo_f14')
      mask Display: disp('?')
  More Info44 : Subsystem
      settings: OpenFcn=showdemo('sldemo_f14')
      mask Display: disp('?')
  More Info45 : Subsystem
      settings: OpenFcn=showdemo('sldemo_f14')
      mask Display: disp('?')
  More Info46 : Subsystem
      settings: OpenFcn=showdemo('sldemo_f14')
      mask Display: disp('?')
  More Info47 : Subsystem
      settings: OpenFcn=showdemo('sldemo_f14')
      mask Display: disp('?')
  More Info48 : Subsystem
      settings: OpenFcn=showdemo('sldemo_f14')
      mask Display: disp('?')
  More Info49 : Subsystem
      settings: OpenFcn=showdemo('sldemo_f14')
      mask Display: disp('?')
  More Info5 : Subsystem
      settings: OpenFcn=showdemo('sldemo_f14')
      mask Display: disp('?')
  More Info50 : Subsystem
      settings: OpenFcn=showdemo('sldemo_f14')
      mask Display: disp('?')
  More Info51 : Subsystem
      settings: OpenFcn=showdemo('sldemo_f14')
      mask Display: disp('?')
  More Info52 : Subsystem
      settings: OpenFcn=showdemo('sldemo_f14')
      mask Display: disp('?')
  More Info53 : Subsystem
      settings: OpenFcn=showdemo('sldemo_f14')
      mask Display: disp('?')
  More Info54 : Subsystem
      settings: OpenFcn=showdemo('sldemo_f14')
      mask Display: disp('?')
  More Info55 : Subsystem
      settings: OpenFcn=showdemo('sldemo_f14')
      mask Display: disp('?')
  More Info56 : Subsystem
      settings: OpenFcn=showdemo('sldemo_f14')
      mask Display: disp('?')
  More Info57 : Subsystem
      settings: OpenFcn=showdemo('sldemo_f14')
      mask Display: disp('?')
  More Info58 : Subsystem
      settings: OpenFcn=showdemo('sldemo_f14')
      mask Display: disp('?')
  More Info59 : Subsystem
      settings: OpenFcn=showdemo('sldemo_f14')
      mask Display: disp('?')
  More Info6 : Subsystem
      settings: OpenFcn=showdemo('sldemo_f14')
      mask Display: disp('?')
  More Info60 : Subsystem
      settings: OpenFcn=showdemo('sldemo_f14')
      mask Display: disp('?')
  More Info61 : Subsystem
      settings: OpenFcn=showdemo('sldemo_f14')
      mask Display: disp('?')
  More Info62 : Subsystem
      settings: OpenFcn=showdemo('sldemo_f14')
      mask Display: disp('?')
  More Info63 : Subsystem
      settings: OpenFcn=showdemo('sldemo_f14')
      mask Display: disp('?')
  More Info64 : Subsystem
      settings: OpenFcn=showdemo('sldemo_f14')
      mask Display: disp('?')
  More Info65 : Subsystem
      settings: OpenFcn=showdemo('sldemo_f14')
      mask Display: disp('?')
  More Info66 : Subsystem
      settings: OpenFcn=showdemo('sldemo_f14')
      mask Display: disp('?')
  More Info67 : Subsystem
      settings: OpenFcn=showdemo('sldemo_f14')
      mask Display: disp('?')
  More Info68 : Subsystem
      settings: OpenFcn=showdemo('sldemo_f14')
      mask Display: disp('?')
  More Info69 : Subsystem
      settings: OpenFcn=showdemo('sldemo_f14')
      mask Display: disp('?')
  More Info7 : Subsystem
      settings: OpenFcn=showdemo('sldemo_f14')
      mask Display: disp('?')
  More Info70 : Subsystem
      settings: OpenFcn=showdemo('sldemo_f14')
      mask Display: disp('?')
  More Info71 : Subsystem
      settings: OpenFcn=showdemo('sldemo_f14')
      mask Display: disp('?')
  More Info72 : Subsystem
      settings: OpenFcn=showdemo('sldemo_f14')
      mask Display: disp('?')
  More Info73 : Subsystem
      settings: OpenFcn=showdemo('sldemo_f14')
      mask Display: disp('?')
  More Info74 : Subsystem
      settings: OpenFcn=showdemo('sldemo_f14')
      mask Display: disp('?')
  More Info75 : Subsystem
      settings: OpenFcn=showdemo('sldemo_f14')
      mask Display: disp('?')
  More Info76 : Subsystem
      settings: OpenFcn=showdemo('sldemo_f14')
      mask Display: disp('?')
  More Info77 : Subsystem
      settings: OpenFcn=showdemo('sldemo_f14')
      mask Display: disp('?')
  More Info78 : Subsystem
      settings: OpenFcn=showdemo('sldemo_f14')
      mask Display: disp('?')
  More Info79 : Subsystem
      settings: OpenFcn=showdemo('sldemo_f14')
      mask Display: disp('?')
  More Info8 : Subsystem
      settings: OpenFcn=showdemo('sldemo_f14')
      mask Display: disp('?')
  More Info80 : Subsystem
      settings: OpenFcn=showdemo('sldemo_f14')
      mask Display: disp('?')
  More Info81 : Subsystem
      settings: OpenFcn=showdemo('sldemo_f14')
      mask Display: disp('?')
  More Info82 : Subsystem
      settings: OpenFcn=showdemo('sldemo_f14')
      mask Display: disp('?')
  More Info83 : Subsystem
      settings: OpenFcn=showdemo('sldemo_f14')
      mask Display: disp('?')
  More Info84 : Subsystem
      settings: OpenFcn=showdemo('sldemo_f14')
      mask Display: disp('?')
  More Info85 : Subsystem
      settings: OpenFcn=showdemo('sldemo_f14')
      mask Display: disp('?')
  More Info86 : Subsystem
      settings: OpenFcn=showdemo('sldemo_f14')
      mask Display: disp('?')
  More Info87 : Subsystem
      settings: OpenFcn=showdemo('sldemo_f14')
      mask Display: disp('?')
  More Info88 : Subsystem
      settings: OpenFcn=showdemo('sldemo_f14')
      mask Display: disp('?')
  More Info89 : Subsystem
      settings: OpenFcn=showdemo('sldemo_f14')
      mask Display: disp('?')
  More Info9 : Subsystem
      settings: OpenFcn=showdemo('sldemo_f14')
      mask Display: disp('?')
  More Info90 : Subsystem
      settings: OpenFcn=showdemo('sldemo_f14')
      mask Display: disp('?')
  More Info91 : Subsystem
      settings: OpenFcn=showdemo('sldemo_f14')
      mask Display: disp('?')
  More Info92 : Subsystem
      settings: OpenFcn=showdemo('sldemo_f14')
      mask Display: disp('?')
  More Info93 : Subsystem
      settings: OpenFcn=showdemo('sldemo_f14')
      mask Display: disp('?')
  More Info94 : Subsystem
      settings: OpenFcn=showdemo('sldemo_f14')
      mask Display: disp('?')
  More Info95 : Subsystem
      settings: OpenFcn=showdemo('sldemo_f14')
      mask Display: disp('?')
  More Info96 : Subsystem
      settings: OpenFcn=showdemo('sldemo_f14')
      mask Display: disp('?')
  More Info97 : Subsystem
      settings: OpenFcn=showdemo('sldemo_f14')
      mask Display: disp('?')
  More Info98 : Subsystem
      settings: OpenFcn=showdemo('sldemo_f14')
      mask Display: disp('?')
  More Info99 : Subsystem
      settings: OpenFcn=showdemo('sldemo_f14')
      mask Display: disp('?')
  Nz pilot calculation : Subsystem
  Nz pilot calculation1 : Subsystem
  Nz pilot calculation10 : Subsystem
  Nz pilot calculation11 : Subsystem
  Nz pilot calculation12 : Subsystem
  Nz pilot calculation13 : Subsystem
  Nz pilot calculation14 : Subsystem
  Nz pilot calculation15 : Subsystem
  Nz pilot calculation16 : Subsystem
  Nz pilot calculation17 : Subsystem
  Nz pilot calculation18 : Subsystem
  Nz pilot calculation19 : Subsystem
  Nz pilot calculation2 : Subsystem
  Nz pilot calculation20 : Subsystem
  Nz pilot calculation21 : Subsystem
  Nz pilot calculation22 : Subsystem
  Nz pilot calculation23 : Subsystem
  Nz pilot calculation24 : Subsystem
  Nz pilot calculation25 : Subsystem
  Nz pilot calculation26 : Subsystem
  Nz pilot calculation27 : Subsystem
  Nz pilot calculation28 : Subsystem
  Nz pilot calculation29 : Subsystem
  Nz pilot calculation3 : Subsystem
  Nz pilot calculation30 : Subsystem
  Nz pilot calculation31 : Subsystem
  Nz pilot calculation32 : Subsystem
  Nz pilot calculation33 : Subsystem
  Nz pilot calculation34 : Subsystem
  Nz pilot calculation35 : Subsystem
  Nz pilot calculation36 : Subsystem
  Nz pilot calculation37 : Subsystem
  Nz pilot calculation38 : Subsystem
  Nz pilot calculation39 : Subsystem
  Nz pilot calculation4 : Subsystem
  Nz pilot calculation40 : Subsystem
  Nz pilot calculation41 : Subsystem
  Nz pilot calculation42 : Subsystem
  Nz pilot calculation43 : Subsystem
  Nz pilot calculation44 : Subsystem
  Nz pilot calculation45 : Subsystem
  Nz pilot calculation46 : Subsystem
  Nz pilot calculation47 : Subsystem
  Nz pilot calculation48 : Subsystem
  Nz pilot calculation49 : Subsystem
  Nz pilot calculation5 : Subsystem
  Nz pilot calculation50 : Subsystem
  Nz pilot calculation51 : Subsystem
  Nz pilot calculation52 : Subsystem
  Nz pilot calculation53 : Subsystem
  Nz pilot calculation54 : Subsystem
  Nz pilot calculation55 : Subsystem
  Nz pilot calculation56 : Subsystem
  Nz pilot calculation57 : Subsystem
  Nz pilot calculation58 : Subsystem
  Nz pilot calculation59 : Subsystem
  Nz pilot calculation6 : Subsystem
  Nz pilot calculation60 : Subsystem
  Nz pilot calculation61 : Subsystem
  Nz pilot calculation62 : Subsystem
  Nz pilot calculation63 : Subsystem
  Nz pilot calculation64 : Subsystem
  Nz pilot calculation65 : Subsystem
  Nz pilot calculation66 : Subsystem
  Nz pilot calculation67 : Subsystem
  Nz pilot calculation68 : Subsystem
  Nz pilot calculation69 : Subsystem
  Nz pilot calculation7 : Subsystem
  Nz pilot calculation70 : Subsystem
  Nz pilot calculation71 : Subsystem
  Nz pilot calculation72 : Subsystem
  Nz pilot calculation73 : Subsystem
  Nz pilot calculation74 : Subsystem
  Nz pilot calculation75 : Subsystem
  Nz pilot calculation76 : Subsystem
  Nz pilot calculation77 : Subsystem
  Nz pilot calculation78 : Subsystem
  Nz pilot calculation79 : Subsystem
  Nz pilot calculation8 : Subsystem
  Nz pilot calculation80 : Subsystem
  Nz pilot calculation81 : Subsystem
  Nz pilot calculation82 : Subsystem
  Nz pilot calculation83 : Subsystem
  Nz pilot calculation84 : Subsystem
  Nz pilot calculation85 : Subsystem
  Nz pilot calculation86 : Subsystem
  Nz pilot calculation87 : Subsystem
  Nz pilot calculation88 : Subsystem
  Nz pilot calculation89 : Subsystem
  Nz pilot calculation9 : Subsystem
  Nz pilot calculation90 : Subsystem
  Nz pilot calculation91 : Subsystem
  Nz pilot calculation92 : Subsystem
  Nz pilot calculation93 : Subsystem
  Nz pilot calculation94 : Subsystem
  Nz pilot calculation95 : Subsystem
  Nz pilot calculation96 : Subsystem
  Nz pilot calculation97 : Subsystem
  Nz pilot calculation98 : Subsystem
  Nz pilot calculation99 : Subsystem
  Pilot{,1..99} (100 alike) : SignalGenerator  WaveForm=square  Frequency=0.500000  Units=rad/sec
  Pilot G force Scope{,1..99} (100 alike) : Scope
  Stick Input{,1..99} (100 alike) : Scope
  Sum{,1..199} (200 alike) : Sum  Inputs=|++  InputSameDT=on  SaturateOnIntegerOverflow=on  OutDataTypeStr=Inherit: Same as first input
  alpha (rad) : Outport  InitialOutput=0
  Nz Pilot (g) : Outport  Port=2  InitialOutput=0
  alpha (rad)1 : Outport  Port=3  InitialOutput=0
  Nz Pilot (g)1 : Outport  Port=4  InitialOutput=0
  alpha (rad)2 : Outport  Port=5  InitialOutput=0
  Nz Pilot (g)2 : Outport  Port=6  InitialOutput=0
  alpha (rad)3 : Outport  Port=7  InitialOutput=0
  Nz Pilot (g)3 : Outport  Port=8  InitialOutput=0
  alpha (rad)4 : Outport  Port=9  InitialOutput=0
  Nz Pilot (g)4 : Outport  Port=10  InitialOutput=0
  alpha (rad)5 : Outport  Port=11  InitialOutput=0
  Nz Pilot (g)5 : Outport  Port=12  InitialOutput=0
  alpha (rad)6 : Outport  Port=13  InitialOutput=0
  Nz Pilot (g)6 : Outport  Port=14  InitialOutput=0
  alpha (rad)7 : Outport  Port=15  InitialOutput=0
  Nz Pilot (g)7 : Outport  Port=16  InitialOutput=0
  alpha (rad)8 : Outport  Port=17  InitialOutput=0
  Nz Pilot (g)8 : Outport  Port=18  InitialOutput=0
  alpha (rad)9 : Outport  Port=19  InitialOutput=0
  Nz Pilot (g)9 : Outport  Port=20  InitialOutput=0
  alpha (rad)10 : Outport  Port=21  InitialOutput=0
  Nz Pilot (g)10 : Outport  Port=22  InitialOutput=0
  alpha (rad)11 : Outport  Port=23  InitialOutput=0
  Nz Pilot (g)11 : Outport  Port=24  InitialOutput=0
  alpha (rad)12 : Outport  Port=25  InitialOutput=0
  Nz Pilot (g)12 : Outport  Port=26  InitialOutput=0
  alpha (rad)13 : Outport  Port=27  InitialOutput=0
  Nz Pilot (g)13 : Outport  Port=28  InitialOutput=0
  alpha (rad)14 : Outport  Port=29  InitialOutput=0
  Nz Pilot (g)14 : Outport  Port=30  InitialOutput=0
  alpha (rad)15 : Outport  Port=31  InitialOutput=0
  Nz Pilot (g)15 : Outport  Port=32  InitialOutput=0
  alpha (rad)16 : Outport  Port=33  InitialOutput=0
  Nz Pilot (g)16 : Outport  Port=34  InitialOutput=0
  alpha (rad)17 : Outport  Port=35  InitialOutput=0
  Nz Pilot (g)17 : Outport  Port=36  InitialOutput=0
  alpha (rad)18 : Outport  Port=37  InitialOutput=0
  Nz Pilot (g)18 : Outport  Port=38  InitialOutput=0
  alpha (rad)19 : Outport  Port=39  InitialOutput=0
  Nz Pilot (g)19 : Outport  Port=40  InitialOutput=0
  alpha (rad)20 : Outport  Port=41  InitialOutput=0
  Nz Pilot (g)20 : Outport  Port=42  InitialOutput=0
  alpha (rad)21 : Outport  Port=43  InitialOutput=0
  Nz Pilot (g)21 : Outport  Port=44  InitialOutput=0
  alpha (rad)22 : Outport  Port=45  InitialOutput=0
  Nz Pilot (g)22 : Outport  Port=46  InitialOutput=0
  alpha (rad)23 : Outport  Port=47  InitialOutput=0
  Nz Pilot (g)23 : Outport  Port=48  InitialOutput=0
  alpha (rad)24 : Outport  Port=49  InitialOutput=0
  Nz Pilot (g)24 : Outport  Port=50  InitialOutput=0
  alpha (rad)25 : Outport  Port=51  InitialOutput=0
  Nz Pilot (g)25 : Outport  Port=52  InitialOutput=0
  alpha (rad)26 : Outport  Port=53  InitialOutput=0
  Nz Pilot (g)26 : Outport  Port=54  InitialOutput=0
  alpha (rad)27 : Outport  Port=55  InitialOutput=0
  Nz Pilot (g)27 : Outport  Port=56  InitialOutput=0
  alpha (rad)28 : Outport  Port=57  InitialOutput=0
  Nz Pilot (g)28 : Outport  Port=58  InitialOutput=0
  alpha (rad)29 : Outport  Port=59  InitialOutput=0
  Nz Pilot (g)29 : Outport  Port=60  InitialOutput=0
  alpha (rad)30 : Outport  Port=61  InitialOutput=0
  Nz Pilot (g)30 : Outport  Port=62  InitialOutput=0
  alpha (rad)31 : Outport  Port=63  InitialOutput=0
  Nz Pilot (g)31 : Outport  Port=64  InitialOutput=0
  alpha (rad)32 : Outport  Port=65  InitialOutput=0
  Nz Pilot (g)32 : Outport  Port=66  InitialOutput=0
  alpha (rad)33 : Outport  Port=67  InitialOutput=0
  Nz Pilot (g)33 : Outport  Port=68  InitialOutput=0
  alpha (rad)34 : Outport  Port=69  InitialOutput=0
  Nz Pilot (g)34 : Outport  Port=70  InitialOutput=0
  alpha (rad)35 : Outport  Port=71  InitialOutput=0
  Nz Pilot (g)35 : Outport  Port=72  InitialOutput=0
  alpha (rad)36 : Outport  Port=73  InitialOutput=0
  Nz Pilot (g)36 : Outport  Port=74  InitialOutput=0
  alpha (rad)37 : Outport  Port=75  InitialOutput=0
  Nz Pilot (g)37 : Outport  Port=76  InitialOutput=0
  alpha (rad)38 : Outport  Port=77  InitialOutput=0
  Nz Pilot (g)38 : Outport  Port=78  InitialOutput=0
  alpha (rad)39 : Outport  Port=79  InitialOutput=0
  Nz Pilot (g)39 : Outport  Port=80  InitialOutput=0
  alpha (rad)40 : Outport  Port=81  InitialOutput=0
  Nz Pilot (g)40 : Outport  Port=82  InitialOutput=0
  alpha (rad)41 : Outport  Port=83  InitialOutput=0
  Nz Pilot (g)41 : Outport  Port=84  InitialOutput=0
  alpha (rad)42 : Outport  Port=85  InitialOutput=0
  Nz Pilot (g)42 : Outport  Port=86  InitialOutput=0
  alpha (rad)43 : Outport  Port=87  InitialOutput=0
  Nz Pilot (g)43 : Outport  Port=88  InitialOutput=0
  alpha (rad)44 : Outport  Port=89  InitialOutput=0
  Nz Pilot (g)44 : Outport  Port=90  InitialOutput=0
  alpha (rad)45 : Outport  Port=91  InitialOutput=0
  Nz Pilot (g)45 : Outport  Port=92  InitialOutput=0
  alpha (rad)46 : Outport  Port=93  InitialOutput=0
  Nz Pilot (g)46 : Outport  Port=94  InitialOutput=0
  alpha (rad)47 : Outport  Port=95  InitialOutput=0
  Nz Pilot (g)47 : Outport  Port=96  InitialOutput=0
  alpha (rad)48 : Outport  Port=97  InitialOutput=0
  Nz Pilot (g)48 : Outport  Port=98  InitialOutput=0
  alpha (rad)49 : Outport  Port=99  InitialOutput=0
  Nz Pilot (g)49 : Outport  Port=100  InitialOutput=0
  alpha (rad)50 : Outport  Port=101  InitialOutput=0
  Nz Pilot (g)50 : Outport  Port=102  InitialOutput=0
  alpha (rad)51 : Outport  Port=103  InitialOutput=0
  Nz Pilot (g)51 : Outport  Port=104  InitialOutput=0
  alpha (rad)52 : Outport  Port=105  InitialOutput=0
  Nz Pilot (g)52 : Outport  Port=106  InitialOutput=0
  alpha (rad)53 : Outport  Port=107  InitialOutput=0
  Nz Pilot (g)53 : Outport  Port=108  InitialOutput=0
  alpha (rad)54 : Outport  Port=109  InitialOutput=0
  Nz Pilot (g)54 : Outport  Port=110  InitialOutput=0
  alpha (rad)55 : Outport  Port=111  InitialOutput=0
  Nz Pilot (g)55 : Outport  Port=112  InitialOutput=0
  alpha (rad)56 : Outport  Port=113  InitialOutput=0
  Nz Pilot (g)56 : Outport  Port=114  InitialOutput=0
  alpha (rad)57 : Outport  Port=115  InitialOutput=0
  Nz Pilot (g)57 : Outport  Port=116  InitialOutput=0
  alpha (rad)58 : Outport  Port=117  InitialOutput=0
  Nz Pilot (g)58 : Outport  Port=118  InitialOutput=0
  alpha (rad)59 : Outport  Port=119  InitialOutput=0
  Nz Pilot (g)59 : Outport  Port=120  InitialOutput=0
  alpha (rad)60 : Outport  Port=121  InitialOutput=0
  Nz Pilot (g)60 : Outport  Port=122  InitialOutput=0
  alpha (rad)61 : Outport  Port=123  InitialOutput=0
  Nz Pilot (g)61 : Outport  Port=124  InitialOutput=0
  alpha (rad)62 : Outport  Port=125  InitialOutput=0
  Nz Pilot (g)62 : Outport  Port=126  InitialOutput=0
  alpha (rad)63 : Outport  Port=127  InitialOutput=0
  Nz Pilot (g)63 : Outport  Port=128  InitialOutput=0
  alpha (rad)64 : Outport  Port=129  InitialOutput=0
  Nz Pilot (g)64 : Outport  Port=130  InitialOutput=0
  alpha (rad)65 : Outport  Port=131  InitialOutput=0
  Nz Pilot (g)65 : Outport  Port=132  InitialOutput=0
  alpha (rad)66 : Outport  Port=133  InitialOutput=0
  Nz Pilot (g)66 : Outport  Port=134  InitialOutput=0
  alpha (rad)67 : Outport  Port=135  InitialOutput=0
  Nz Pilot (g)67 : Outport  Port=136  InitialOutput=0
  alpha (rad)68 : Outport  Port=137  InitialOutput=0
  Nz Pilot (g)68 : Outport  Port=138  InitialOutput=0
  alpha (rad)69 : Outport  Port=139  InitialOutput=0
  Nz Pilot (g)69 : Outport  Port=140  InitialOutput=0
  alpha (rad)70 : Outport  Port=141  InitialOutput=0
  Nz Pilot (g)70 : Outport  Port=142  InitialOutput=0
  alpha (rad)71 : Outport  Port=143  InitialOutput=0
  Nz Pilot (g)71 : Outport  Port=144  InitialOutput=0
  alpha (rad)72 : Outport  Port=145  InitialOutput=0
  Nz Pilot (g)72 : Outport  Port=146  InitialOutput=0
  alpha (rad)73 : Outport  Port=147  InitialOutput=0
  Nz Pilot (g)73 : Outport  Port=148  InitialOutput=0
  alpha (rad)74 : Outport  Port=149  InitialOutput=0
  Nz Pilot (g)74 : Outport  Port=150  InitialOutput=0
  alpha (rad)75 : Outport  Port=151  InitialOutput=0
  Nz Pilot (g)75 : Outport  Port=152  InitialOutput=0
  alpha (rad)76 : Outport  Port=153  InitialOutput=0
  Nz Pilot (g)76 : Outport  Port=154  InitialOutput=0
  alpha (rad)77 : Outport  Port=155  InitialOutput=0
  Nz Pilot (g)77 : Outport  Port=156  InitialOutput=0
  alpha (rad)78 : Outport  Port=157  InitialOutput=0
  Nz Pilot (g)78 : Outport  Port=158  InitialOutput=0
  alpha (rad)79 : Outport  Port=159  InitialOutput=0
  Nz Pilot (g)79 : Outport  Port=160  InitialOutput=0
  alpha (rad)80 : Outport  Port=161  InitialOutput=0
  Nz Pilot (g)80 : Outport  Port=162  InitialOutput=0
  alpha (rad)81 : Outport  Port=163  InitialOutput=0
  Nz Pilot (g)81 : Outport  Port=164  InitialOutput=0
  alpha (rad)82 : Outport  Port=165  InitialOutput=0
  Nz Pilot (g)82 : Outport  Port=166  InitialOutput=0
  alpha (rad)83 : Outport  Port=167  InitialOutput=0
  Nz Pilot (g)83 : Outport  Port=168  InitialOutput=0
  alpha (rad)84 : Outport  Port=169  InitialOutput=0
  Nz Pilot (g)84 : Outport  Port=170  InitialOutput=0
  alpha (rad)85 : Outport  Port=171  InitialOutput=0
  Nz Pilot (g)85 : Outport  Port=172  InitialOutput=0
  alpha (rad)86 : Outport  Port=173  InitialOutput=0
  Nz Pilot (g)86 : Outport  Port=174  InitialOutput=0
  alpha (rad)87 : Outport  Port=175  InitialOutput=0
  Nz Pilot (g)87 : Outport  Port=176  InitialOutput=0
  alpha (rad)88 : Outport  Port=177  InitialOutput=0
  Nz Pilot (g)88 : Outport  Port=178  InitialOutput=0
  alpha (rad)89 : Outport  Port=179  InitialOutput=0
  Nz Pilot (g)89 : Outport  Port=180  InitialOutput=0
  alpha (rad)90 : Outport  Port=181  InitialOutput=0
  Nz Pilot (g)90 : Outport  Port=182  InitialOutput=0
  alpha (rad)91 : Outport  Port=183  InitialOutput=0
  Nz Pilot (g)91 : Outport  Port=184  InitialOutput=0
  alpha (rad)92 : Outport  Port=185  InitialOutput=0
  Nz Pilot (g)92 : Outport  Port=186  InitialOutput=0
  alpha (rad)93 : Outport  Port=187  InitialOutput=0
  Nz Pilot (g)93 : Outport  Port=188  InitialOutput=0
  alpha (rad)94 : Outport  Port=189  InitialOutput=0
  Nz Pilot (g)94 : Outport  Port=190  InitialOutput=0
  alpha (rad)95 : Outport  Port=191  InitialOutput=0
  Nz Pilot (g)95 : Outport  Port=192  InitialOutput=0
  alpha (rad)96 : Outport  Port=193  InitialOutput=0
  Nz Pilot (g)96 : Outport  Port=194  InitialOutput=0
  alpha (rad)97 : Outport  Port=195  InitialOutput=0
  Nz Pilot (g)97 : Outport  Port=196  InitialOutput=0
  alpha (rad)98 : Outport  Port=197  InitialOutput=0
  Nz Pilot (g)98 : Outport  Port=198  InitialOutput=0
  alpha (rad)99 : Outport  Port=199  InitialOutput=0
  Nz Pilot (g)99 : Outport  Port=200  InitialOutput=0
  wires:
  Gain5/1 -> alpha (rad)/1, Angle of Attack/1, Controller/2(alpha (rad))
  Aircraft Dynamics Model/1(Vertical Velocity w (ft/sec)) -> Gain5/1, Nz pilot calculation/1(w)  "w"
  Nz pilot calculation/1(Pilot g force (g)) -> Pilot G force Scope/1, Nz Pilot (g)/1
  Gain2/1 -> Sum/1
  Gain/1 -> Aircraft Dynamics Model/2(Vertical Gust wGust (ft/sec))
  Pilot/1 -> Sum1/1
  u/1 -> Sum1/2
  Dryden Wind Gust Models/2(Qg) -> Gain1/1  "qGust"
  Dryden Wind Gust Models/1(Wg) -> Gain2/1, Gain/1  "wGust"
  Sum/1 -> Aircraft Dynamics Model/3(Rotary Gust qGust (rad/sec))
  Gain1/1 -> Sum/2
  Aircraft Dynamics Model/2(Pitch Rate q (rad/sec)) -> Nz pilot calculation/2(q), Controller/3(q (rad/sec))  "q"
  Actuator Model/1 -> Aircraft Dynamics Model/1(Elevator Deflection d (deg))
  Controller/1(Elevator Command (deg)) -> Actuator Model/1
  Sum1/1 -> Stick Input/1, Controller/1(Stick Input (in))
  u1/1 -> Sum3/2
  Sum2/1 -> Aircraft Dynamics Model1/3(Rotary Gust qGust (rad/sec))
  Gain7/1 -> alpha (rad)1/1, Angle of Attack1/1, Controller1/2(alpha (rad))
  Dryden Wind Gust Models1/2(Qg) -> Gain4/1  "qGust"
  Actuator Model1/1 -> Aircraft Dynamics Model1/1(Elevator Deflection d (deg))
  Aircraft Dynamics Model1/2(Pitch Rate q (rad/sec)) -> Nz pilot calculation1/2(q), Controller1/3(q (rad/sec))  "q"
  Pilot1/1 -> Sum3/1
  Gain3/1 -> Aircraft Dynamics Model1/2(Vertical Gust wGust (ft/sec))
  Aircraft Dynamics Model1/1(Vertical Velocity w (ft/sec)) -> Gain7/1, Nz pilot calculation1/1(w)  "w"
  Sum3/1 -> Stick Input1/1, Controller1/1(Stick Input (in))
  Gain4/1 -> Sum2/2
  Controller1/1(Elevator Command (deg)) -> Actuator Model1/1
  Dryden Wind Gust Models1/1(Wg) -> Gain6/1, Gain3/1  "wGust"
  Gain6/1 -> Sum2/1
  Nz pilot calculation1/1(Pilot g force (g)) -> Pilot G force Scope1/1, Nz Pilot (g)1/1
  u2/1 -> Sum5/2
  Sum4/1 -> Aircraft Dynamics Model2/3(Rotary Gust qGust (rad/sec))
  Gain11/1 -> alpha (rad)2/1, Angle of Attack2/1, Controller2/2(alpha (rad))
  Dryden Wind Gust Models2/2(Qg) -> Gain9/1  "qGust"
  Actuator Model2/1 -> Aircraft Dynamics Model2/1(Elevator Deflection d (deg))
  Aircraft Dynamics Model2/2(Pitch Rate q (rad/sec)) -> Nz pilot calculation2/2(q), Controller2/3(q (rad/sec))  "q"
  Pilot2/1 -> Sum5/1
  Gain8/1 -> Aircraft Dynamics Model2/2(Vertical Gust wGust (ft/sec))
  Aircraft Dynamics Model2/1(Vertical Velocity w (ft/sec)) -> Gain11/1, Nz pilot calculation2/1(w)  "w"
  Sum5/1 -> Stick Input2/1, Controller2/1(Stick Input (in))
  Gain9/1 -> Sum4/2
  Controller2/1(Elevator Command (deg)) -> Actuator Model2/1
  Dryden Wind Gust Models2/1(Wg) -> Gain10/1, Gain8/1  "wGust"
  Gain10/1 -> Sum4/1
  Nz pilot calculation2/1(Pilot g force (g)) -> Pilot G force Scope2/1, Nz Pilot (g)2/1
  Gain15/1 -> Aircraft Dynamics Model4/2(Vertical Gust wGust (ft/sec))
  Sum8/1 -> Aircraft Dynamics Model4/3(Rotary Gust qGust (rad/sec))
  Gain18/1 -> Sum8/1
  Gain16/1 -> Sum8/2
  Dryden Wind Gust Models4/1(Wg) -> Gain18/1, Gain15/1  "wGust"
  Controller4/1(Elevator Command (deg)) -> Actuator Model4/1
  Aircraft Dynamics Model4/2(Pitch Rate q (rad/sec)) -> Nz pilot calculation4/2(q), Controller4/3(q (rad/sec))  "q"
  u3/1 -> Sum7/2
  u4/1 -> Sum9/2
  Sum6/1 -> Aircraft Dynamics Model3/3(Rotary Gust qGust (rad/sec))
  Gain17/1 -> alpha (rad)3/1, Angle of Attack3/1, Controller3/2(alpha (rad))
  Dryden Wind Gust Models3/2(Qg) -> Gain13/1  "qGust"
  Actuator Model3/1 -> Aircraft Dynamics Model3/1(Elevator Deflection d (deg))
  Aircraft Dynamics Model3/2(Pitch Rate q (rad/sec)) -> Nz pilot calculation3/2(q), Controller3/3(q (rad/sec))  "q"
  Pilot3/1 -> Sum7/1
  Gain12/1 -> Aircraft Dynamics Model3/2(Vertical Gust wGust (ft/sec))
  Actuator Model4/1 -> Aircraft Dynamics Model4/1(Elevator Deflection d (deg))
  Aircraft Dynamics Model4/1(Vertical Velocity w (ft/sec)) -> Gain19/1, Nz pilot calculation4/1(w)  "w"
  Sum9/1 -> Stick Input4/1, Controller4/1(Stick Input (in))
  Pilot4/1 -> Sum9/1
  Aircraft Dynamics Model3/1(Vertical Velocity w (ft/sec)) -> Gain17/1, Nz pilot calculation3/1(w)  "w"
  Nz pilot calculation4/1(Pilot g force (g)) -> Pilot G force Scope4/1, Nz Pilot (g)4/1
  Sum7/1 -> Stick Input3/1, Controller3/1(Stick Input (in))
  Gain13/1 -> Sum6/2
  Controller3/1(Elevator Command (deg)) -> Actuator Model3/1
  Gain19/1 -> alpha (rad)4/1, Angle of Attack4/1, Controller4/2(alpha (rad))
  Dryden Wind Gust Models3/1(Wg) -> Gain14/1, Gain12/1  "wGust"
  Dryden Wind Gust Models4/2(Qg) -> Gain16/1  "qGust"
  Gain14/1 -> Sum6/1
  Nz pilot calculation3/1(Pilot g force (g)) -> Pilot G force Scope3/1, Nz Pilot (g)3/1
  Gain33/1 -> Aircraft Dynamics Model6/2(Vertical Gust wGust (ft/sec))
  Aircraft Dynamics Model6/1(Vertical Velocity w (ft/sec)) -> Gain37/1, Nz pilot calculation6/1(w)  "w"
  Dryden Wind Gust Models6/2(Qg) -> Gain34/1  "qGust"
  Actuator Model6/1 -> Aircraft Dynamics Model6/1(Elevator Deflection d (deg))
  Sum12/1 -> Aircraft Dynamics Model6/3(Rotary Gust qGust (rad/sec))
  u6/1 -> Sum13/2
  Pilot6/1 -> Sum13/1
  Gain34/1 -> Sum12/2
  Nz pilot calculation6/1(Pilot g force (g)) -> Pilot G force Scope6/1, Nz Pilot (g)6/1
  Dryden Wind Gust Models6/1(Wg) -> Gain36/1, Gain33/1  "wGust"
  Controller6/1(Elevator Command (deg)) -> Actuator Model6/1
  u5/1 -> Sum11/2
  Sum10/1 -> Aircraft Dynamics Model5/3(Rotary Gust qGust (rad/sec))
  Gain21/1 -> Sum10/2
  Gain35/1 -> alpha (rad)5/1, Angle of Attack5/1, Controller5/2(alpha (rad))
  Dryden Wind Gust Models5/2(Qg) -> Gain21/1  "qGust"
  Actuator Model5/1 -> Aircraft Dynamics Model5/1(Elevator Deflection d (deg))
  Aircraft Dynamics Model5/2(Pitch Rate q (rad/sec)) -> Nz pilot calculation5/2(q), Controller5/3(q (rad/sec))  "q"
  Pilot5/1 -> Sum11/1
  Gain20/1 -> Aircraft Dynamics Model5/2(Vertical Gust wGust (ft/sec))
  Sum13/1 -> Stick Input6/1, Controller6/1(Stick Input (in))
  Aircraft Dynamics Model5/1(Vertical Velocity w (ft/sec)) -> Gain35/1, Nz pilot calculation5/1(w)  "w"
  Nz pilot calculation7/1(Pilot g force (g)) -> Pilot G force Scope7/1, Nz Pilot (g)7/1
  Gain22/1 -> Sum14/1
  Dryden Wind Gust Models7/1(Wg) -> Gain22/1, Gain38/1  "wGust"
  Controller7/1(Elevator Command (deg)) -> Actuator Model7/1
  Gain39/1 -> Sum14/2
  Sum15/1 -> Stick Input7/1, Controller7/1(Stick Input (in))
  Gain36/1 -> Sum12/1
  Pilot7/1 -> Sum15/1
  Gain38/1 -> Aircraft Dynamics Model7/2(Vertical Gust wGust (ft/sec))
  Aircraft Dynamics Model7/1(Vertical Velocity w (ft/sec)) -> Gain23/1, Nz pilot calculation7/1(w)  "w"
  Aircraft Dynamics Model7/2(Pitch Rate q (rad/sec)) -> Nz pilot calculation7/2(q), Controller7/3(q (rad/sec))  "q"
  Gain23/1 -> alpha (rad)7/1, Angle of Attack7/1, Controller7/2(alpha (rad))
  Dryden Wind Gust Models7/2(Qg) -> Gain39/1  "qGust"
  Sum14/1 -> Aircraft Dynamics Model7/3(Rotary Gust qGust (rad/sec))
  u7/1 -> Sum15/2
  Gain31/1 -> alpha (rad)9/1, Angle of Attack9/1, Controller9/2(alpha (rad))
  Dryden Wind Gust Models9/2(Qg) -> Gain28/1  "qGust"
  Sum11/1 -> Stick Input5/1, Controller5/1(Stick Input (in))
  Sum19/1 -> Stick Input9/1, Controller9/1(Stick Input (in))
  Nz pilot calculation9/1(Pilot g force (g)) -> Pilot G force Scope9/1, Nz Pilot (g)9/1
  Actuator Model7/1 -> Aircraft Dynamics Model7/1(Elevator Deflection d (deg))
  Gain25/1 -> Sum16/2
  Pilot9/1 -> Sum19/1
  Sum17/1 -> Stick Input8/1, Controller8/1(Stick Input (in))
  Controller8/1(Elevator Command (deg)) -> Actuator Model8/1
  Aircraft Dynamics Model9/1(Vertical Velocity w (ft/sec)) -> Gain31/1, Nz pilot calculation9/1(w)  "w"
  Aircraft Dynamics Model8/2(Pitch Rate q (rad/sec)) -> Nz pilot calculation8/2(q), Controller8/3(q (rad/sec))  "q"
  Aircraft Dynamics Model8/1(Vertical Velocity w (ft/sec)) -> Gain29/1, Nz pilot calculation8/1(w)  "w"
  Dryden Wind Gust Models8/2(Qg) -> Gain25/1  "qGust"
  Pilot8/1 -> Sum17/1
  Actuator Model8/1 -> Aircraft Dynamics Model8/1(Elevator Deflection d (deg))
  Dryden Wind Gust Models8/1(Wg) -> Gain26/1, Gain24/1  "wGust"
  Actuator Model9/1 -> Aircraft Dynamics Model9/1(Elevator Deflection d (deg))
  Nz pilot calculation8/1(Pilot g force (g)) -> Pilot G force Scope8/1, Nz Pilot (g)8/1
  Gain26/1 -> Sum16/1
  Gain24/1 -> Aircraft Dynamics Model8/2(Vertical Gust wGust (ft/sec))
  Gain29/1 -> alpha (rad)8/1, Angle of Attack8/1, Controller8/2(alpha (rad))
  Controller9/1(Elevator Command (deg)) -> Actuator Model9/1
  Gain30/1 -> Sum18/1
  Aircraft Dynamics Model9/2(Pitch Rate q (rad/sec)) -> Nz pilot calculation9/2(q), Controller9/3(q (rad/sec))  "q"
  Gain27/1 -> Aircraft Dynamics Model9/2(Vertical Gust wGust (ft/sec))
  u8/1 -> Sum17/2
  Dryden Wind Gust Models9/1(Wg) -> Gain30/1, Gain27/1  "wGust"
  Sum18/1 -> Aircraft Dynamics Model9/3(Rotary Gust qGust (rad/sec))
  Controller5/1(Elevator Command (deg)) -> Actuator Model5/1
  Sum16/1 -> Aircraft Dynamics Model8/3(Rotary Gust qGust (rad/sec))
  Gain37/1 -> alpha (rad)6/1, Angle of Attack6/1, Controller6/2(alpha (rad))
  Dryden Wind Gust Models5/1(Wg) -> Gain32/1, Gain20/1  "wGust"
  Aircraft Dynamics Model6/2(Pitch Rate q (rad/sec)) -> Nz pilot calculation6/2(q), Controller6/3(q (rad/sec))  "q"
  Gain32/1 -> Sum10/1
  u9/1 -> Sum19/2
  Gain28/1 -> Sum18/2
  Nz pilot calculation5/1(Pilot g force (g)) -> Pilot G force Scope5/1, Nz Pilot (g)5/1
  Controller18/1(Elevator Command (deg)) -> Actuator Model18/1
  Gain63/1 -> Aircraft Dynamics Model11/2(Vertical Gust wGust (ft/sec))
  Dryden Wind Gust Models11/2(Qg) -> Gain74/1  "qGust"
  Actuator Model11/1 -> Aircraft Dynamics Model11/1(Elevator Deflection d (deg))
  Sum32/1 -> Aircraft Dynamics Model11/3(Rotary Gust qGust (rad/sec))
  Pilot11/1 -> Sum33/1
  Gain74/1 -> Sum32/2
  Nz pilot calculation11/1(Pilot g force (g)) -> Pilot G force Scope11/1, Nz Pilot (g)11/1
  Dryden Wind Gust Models11/1(Wg) -> Gain76/1, Gain63/1  "wGust"
  u10/1 -> Sum21/2
  Sum20/1 -> Aircraft Dynamics Model10/3(Rotary Gust qGust (rad/sec))
  Gain41/1 -> Sum20/2
  Gain75/1 -> alpha (rad)10/1, Angle of Attack10/1, Controller10/2(alpha (rad))
  Dryden Wind Gust Models10/2(Qg) -> Gain41/1  "qGust"
  Aircraft Dynamics Model10/2(Pitch Rate q (rad/sec)) -> Nz pilot calculation10/2(q), Controller10/3(q (rad/sec))  "q"
  Gain61/1 -> Sum30/2
  Dryden Wind Gust Models15/1(Wg) -> Gain66/1, Gain53/1  "wGust"
  Sum28/1 -> Aircraft Dynamics Model18/3(Rotary Gust qGust (rad/sec))
  u11/1 -> Sum33/2
  u18/1 -> Sum29/2
  Controller15/1(Elevator Command (deg)) -> Actuator Model15/1
  Actuator Model10/1 -> Aircraft Dynamics Model10/1(Elevator Deflection d (deg))
  Sum30/1 -> Aircraft Dynamics Model19/3(Rotary Gust qGust (rad/sec))
  Dryden Wind Gust Models19/1(Wg) -> Gain64/1, Gain60/1  "wGust"
  Aircraft Dynamics Model19/2(Pitch Rate q (rad/sec)) -> Nz pilot calculation19/2(q), Controller19/3(q (rad/sec))  "q"
  Gain62/1 -> alpha (rad)18/1, Angle of Attack18/1, Controller18/2(alpha (rad))
  Gain59/1 -> Sum28/1
  Nz pilot calculation18/1(Pilot g force (g)) -> Pilot G force Scope18/1, Nz Pilot (g)18/1
  Actuator Model18/1 -> Aircraft Dynamics Model18/1(Elevator Deflection d (deg))
  Dryden Wind Gust Models18/1(Wg) -> Gain59/1, Gain57/1  "wGust"
  Actuator Model19/1 -> Aircraft Dynamics Model19/1(Elevator Deflection d (deg))
  Pilot18/1 -> Sum29/1
  Aircraft Dynamics Model19/1(Vertical Velocity w (ft/sec)) -> Gain65/1, Nz pilot calculation19/1(w)  "w"
  Aircraft Dynamics Model18/2(Pitch Rate q (rad/sec)) -> Nz pilot calculation18/2(q), Controller18/3(q (rad/sec))  "q"
  Gain40/1 -> Aircraft Dynamics Model10/2(Vertical Gust wGust (ft/sec))
  Dryden Wind Gust Models17/1(Wg) -> Gain55/1, Gain72/1  "wGust"
  Nz pilot calculation15/1(Pilot g force (g)) -> Pilot G force Scope15/1, Nz Pilot (g)15/1
  Nz pilot calculation17/1(Pilot g force (g)) -> Pilot G force Scope17/1, Nz Pilot (g)17/1
  Gain55/1 -> Sum26/1
  Aircraft Dynamics Model18/1(Vertical Velocity w (ft/sec)) -> Gain62/1, Nz pilot calculation18/1(w)  "w"
  Aircraft Dynamics Model15/1(Vertical Velocity w (ft/sec)) -> Gain69/1, Nz pilot calculation15/1(w)  "w"
  Sum26/1 -> Aircraft Dynamics Model17/3(Rotary Gust qGust (rad/sec))
  Gain56/1 -> alpha (rad)17/1, Angle of Attack17/1, Controller17/2(alpha (rad))
  Aircraft Dynamics Model17/2(Pitch Rate q (rad/sec)) -> Nz pilot calculation17/2(q), Controller17/3(q (rad/sec))  "q"
  u17/1 -> Sum27/2
  Gain72/1 -> Aircraft Dynamics Model17/2(Vertical Gust wGust (ft/sec))
  Pilot17/1 -> Sum27/1
  Gain70/1 -> Sum24/1
  Sum27/1 -> Stick Input17/1, Controller17/1(Stick Input (in))
  Aircraft Dynamics Model17/1(Vertical Velocity w (ft/sec)) -> Gain56/1, Nz pilot calculation17/1(w)  "w"
  Sum25/1 -> Stick Input16/1, Controller16/1(Stick Input (in))
  Gain73/1 -> Sum26/2
  u19/1 -> Sum31/2
  Sum23/1 -> Stick Input15/1, Controller15/1(Stick Input (in))
  Sum33/1 -> Stick Input11/1, Controller11/1(Stick Input (in))
  Aircraft Dynamics Model10/1(Vertical Velocity w (ft/sec)) -> Gain75/1, Nz pilot calculation10/1(w)  "w"
  Nz pilot calculation12/1(Pilot g force (g)) -> Pilot G force Scope12/1, Nz Pilot (g)12/1
  Gain79/1 -> Sum34/2
  Sum35/1 -> Stick Input12/1, Controller12/1(Stick Input (in))
  Gain66/1 -> Sum22/1
  Gain76/1 -> Sum32/1
  Pilot12/1 -> Sum35/1
  Gain78/1 -> Aircraft Dynamics Model12/2(Vertical Gust wGust (ft/sec))
  Aircraft Dynamics Model12/1(Vertical Velocity w (ft/sec)) -> Gain43/1, Nz pilot calculation12/1(w)  "w"
  Aircraft Dynamics Model12/2(Pitch Rate q (rad/sec)) -> Nz pilot calculation12/2(q), Controller12/3(q (rad/sec))  "q"
  Gain43/1 -> alpha (rad)12/1, Angle of Attack12/1, Controller12/2(alpha (rad))
  Dryden Wind Gust Models12/2(Qg) -> Gain79/1  "qGust"
  u12/1 -> Sum35/2
  Gain51/1 -> alpha (rad)14/1, Angle of Attack14/1, Controller14/2(alpha (rad))
  Dryden Wind Gust Models14/2(Qg) -> Gain48/1  "qGust"
  Controller13/1(Elevator Command (deg)) -> Actuator Model13/1
  Gain46/1 -> Sum36/1
  Nz pilot calculation13/1(Pilot g force (g)) -> Pilot G force Scope13/1, Nz Pilot (g)13/1
  Sum39/1 -> Stick Input14/1, Controller14/1(Stick Input (in))
  Nz pilot calculation14/1(Pilot g force (g)) -> Pilot G force Scope14/1, Nz Pilot (g)14/1
  Actuator Model12/1 -> Aircraft Dynamics Model12/1(Elevator Deflection d (deg))
  Gain45/1 -> Sum36/2
  Aircraft Dynamics Model13/1(Vertical Velocity w (ft/sec)) -> Gain49/1, Nz pilot calculation13/1(w)  "w"
  Dryden Wind Gust Models17/2(Qg) -> Gain73/1  "qGust"
  Pilot14/1 -> Sum39/1
  Sum37/1 -> Stick Input13/1, Controller13/1(Stick Input (in))
  Aircraft Dynamics Model14/1(Vertical Velocity w (ft/sec)) -> Gain51/1, Nz pilot calculation14/1(w)  "w"
  Dryden Wind Gust Models13/1(Wg) -> Gain46/1, Gain44/1  "wGust"
  Aircraft Dynamics Model13/2(Pitch Rate q (rad/sec)) -> Nz pilot calculation13/2(q), Controller13/3(q (rad/sec))  "q"
  Dryden Wind Gust Models13/2(Qg) -> Gain45/1  "qGust"
  Actuator Model13/1 -> Aircraft Dynamics Model13/1(Elevator Deflection d (deg))
  Sum36/1 -> Aircraft Dynamics Model13/3(Rotary Gust qGust (rad/sec))
  Actuator Model14/1 -> Aircraft Dynamics Model14/1(Elevator Deflection d (deg))
  Gain44/1 -> Aircraft Dynamics Model13/2(Vertical Gust wGust (ft/sec))
  Gain49/1 -> alpha (rad)13/1, Angle of Attack13/1, Controller13/2(alpha (rad))
  Controller14/1(Elevator Command (deg)) -> Actuator Model14/1
  Gain50/1 -> Sum38/1
  Aircraft Dynamics Model14/2(Pitch Rate q (rad/sec)) -> Nz pilot calculation14/2(q), Controller14/3(q (rad/sec))  "q"
  Gain71/1 -> alpha (rad)16/1, Angle of Attack16/1, Controller16/2(alpha (rad))
  Gain47/1 -> Aircraft Dynamics Model14/2(Vertical Gust wGust (ft/sec))
  u14/1 -> Sum39/2
  u13/1 -> Sum37/2
  Controller17/1(Elevator Command (deg)) -> Actuator Model17/1
  Dryden Wind Gust Models14/1(Wg) -> Gain50/1, Gain47/1  "wGust"
  Aircraft Dynamics Model11/2(Pitch Rate q (rad/sec)) -> Nz pilot calculation11/2(q), Controller11/3(q (rad/sec))  "q"
  Sum38/1 -> Aircraft Dynamics Model14/3(Rotary Gust qGust (rad/sec))
  Gain57/1 -> Aircraft Dynamics Model18/2(Vertical Gust wGust (ft/sec))
  Gain53/1 -> Aircraft Dynamics Model15/2(Vertical Gust wGust (ft/sec))
  Pilot15/1 -> Sum23/1
  Gain54/1 -> Sum22/2
  u15/1 -> Sum23/2
  Nz pilot calculation16/1(Pilot g force (g)) -> Pilot G force Scope16/1, Nz Pilot (g)16/1
  Gain42/1 -> Sum34/1
  Dryden Wind Gust Models16/1(Wg) -> Gain70/1, Gain67/1  "wGust"
  Actuator Model16/1 -> Aircraft Dynamics Model16/1(Elevator Deflection d (deg))
  Gain77/1 -> alpha (rad)11/1, Angle of Attack11/1, Controller11/2(alpha (rad))
  Controller10/1(Elevator Command (deg)) -> Actuator Model10/1
  Gain68/1 -> Sum24/2
  Sum24/1 -> Aircraft Dynamics Model16/3(Rotary Gust qGust (rad/sec))
  Aircraft Dynamics Model16/1(Vertical Velocity w (ft/sec)) -> Gain71/1, Nz pilot calculation16/1(w)  "w"
  Dryden Wind Gust Models12/1(Wg) -> Gain42/1, Gain78/1  "wGust"
  Gain67/1 -> Aircraft Dynamics Model16/2(Vertical Gust wGust (ft/sec))
  Dryden Wind Gust Models10/1(Wg) -> Gain52/1, Gain40/1  "wGust"
  Gain69/1 -> alpha (rad)15/1, Angle of Attack15/1, Controller15/2(alpha (rad))
  Gain52/1 -> Sum20/1
  Aircraft Dynamics Model16/2(Pitch Rate q (rad/sec)) -> Nz pilot calculation16/2(q), Controller16/3(q (rad/sec))  "q"
  Nz pilot calculation10/1(Pilot g force (g)) -> Pilot G force Scope10/1, Nz Pilot (g)10/1
  Dryden Wind Gust Models18/2(Qg) -> Gain58/1  "qGust"
  Aircraft Dynamics Model15/2(Pitch Rate q (rad/sec)) -> Nz pilot calculation15/2(q), Controller15/3(q (rad/sec))  "q"
  Gain48/1 -> Sum38/2
  Pilot16/1 -> Sum25/1
  Dryden Wind Gust Models15/2(Qg) -> Gain54/1  "qGust"
  Actuator Model15/1 -> Aircraft Dynamics Model15/1(Elevator Deflection d (deg))
  Pilot13/1 -> Sum37/1
  Controller16/1(Elevator Command (deg)) -> Actuator Model16/1
  Sum22/1 -> Aircraft Dynamics Model15/3(Rotary Gust qGust (rad/sec))
  Gain65/1 -> alpha (rad)19/1, Angle of Attack19/1, Controller19/2(alpha (rad))
  Dryden Wind Gust Models16/2(Qg) -> Gain68/1  "qGust"
  Aircraft Dynamics Model11/1(Vertical Velocity w (ft/sec)) -> Gain77/1, Nz pilot calculation11/1(w)  "w"
  Controller19/1(Elevator Command (deg)) -> Actuator Model19/1
  Controller11/1(Elevator Command (deg)) -> Actuator Model11/1
  Pilot10/1 -> Sum21/1
  Sum31/1 -> Stick Input19/1, Controller19/1(Stick Input (in))
  u16/1 -> Sum25/2
  Sum29/1 -> Stick Input18/1, Controller18/1(Stick Input (in))
  Gain64/1 -> Sum30/1
  Nz pilot calculation19/1(Pilot g force (g)) -> Pilot G force Scope19/1, Nz Pilot (g)19/1
  Gain58/1 -> Sum28/2
  Pilot19/1 -> Sum31/1
  Actuator Model17/1 -> Aircraft Dynamics Model17/1(Elevator Deflection d (deg))
  Sum21/1 -> Stick Input10/1, Controller10/1(Stick Input (in))
  Gain60/1 -> Aircraft Dynamics Model19/2(Vertical Gust wGust (ft/sec))
  Controller12/1(Elevator Command (deg)) -> Actuator Model12/1
  Sum34/1 -> Aircraft Dynamics Model12/3(Rotary Gust qGust (rad/sec))
  Dryden Wind Gust Models19/2(Qg) -> Gain61/1  "qGust"
  Controller28/1(Elevator Command (deg)) -> Actuator Model28/1
  Gain103/1 -> Aircraft Dynamics Model21/2(Vertical Gust wGust (ft/sec))
  Dryden Wind Gust Models21/2(Qg) -> Gain114/1  "qGust"
  Actuator Model21/1 -> Aircraft Dynamics Model21/1(Elevator Deflection d (deg))
  Sum52/1 -> Aircraft Dynamics Model21/3(Rotary Gust qGust (rad/sec))
  Pilot21/1 -> Sum53/1
  Gain114/1 -> Sum52/2
  Nz pilot calculation21/1(Pilot g force (g)) -> Pilot G force Scope21/1, Nz Pilot (g)21/1
  Dryden Wind Gust Models21/1(Wg) -> Gain116/1, Gain103/1  "wGust"
  u20/1 -> Sum41/2
  Sum40/1 -> Aircraft Dynamics Model20/3(Rotary Gust qGust (rad/sec))
  Gain81/1 -> Sum40/2
  Gain115/1 -> alpha (rad)20/1, Angle of Attack20/1, Controller20/2(alpha (rad))
  Dryden Wind Gust Models20/2(Qg) -> Gain81/1  "qGust"
  Aircraft Dynamics Model20/2(Pitch Rate q (rad/sec)) -> Nz pilot calculation20/2(q), Controller20/3(q (rad/sec))  "q"
  Gain101/1 -> Sum50/2
  Dryden Wind Gust Models25/1(Wg) -> Gain106/1, Gain93/1  "wGust"
  Sum48/1 -> Aircraft Dynamics Model28/3(Rotary Gust qGust (rad/sec))
  u21/1 -> Sum53/2
  u28/1 -> Sum49/2
  Controller25/1(Elevator Command (deg)) -> Actuator Model25/1
  Actuator Model20/1 -> Aircraft Dynamics Model20/1(Elevator Deflection d (deg))
  Sum50/1 -> Aircraft Dynamics Model29/3(Rotary Gust qGust (rad/sec))
  Dryden Wind Gust Models29/1(Wg) -> Gain104/1, Gain100/1  "wGust"
  Aircraft Dynamics Model29/2(Pitch Rate q (rad/sec)) -> Nz pilot calculation29/2(q), Controller29/3(q (rad/sec))  "q"
  Gain102/1 -> alpha (rad)28/1, Angle of Attack28/1, Controller28/2(alpha (rad))
  Gain99/1 -> Sum48/1
  Nz pilot calculation28/1(Pilot g force (g)) -> Pilot G force Scope28/1, Nz Pilot (g)28/1
  Actuator Model28/1 -> Aircraft Dynamics Model28/1(Elevator Deflection d (deg))
  Dryden Wind Gust Models28/1(Wg) -> Gain99/1, Gain97/1  "wGust"
  Actuator Model29/1 -> Aircraft Dynamics Model29/1(Elevator Deflection d (deg))
  Pilot28/1 -> Sum49/1
  Aircraft Dynamics Model29/1(Vertical Velocity w (ft/sec)) -> Gain105/1, Nz pilot calculation29/1(w)  "w"
  Aircraft Dynamics Model28/2(Pitch Rate q (rad/sec)) -> Nz pilot calculation28/2(q), Controller28/3(q (rad/sec))  "q"
  Gain80/1 -> Aircraft Dynamics Model20/2(Vertical Gust wGust (ft/sec))
  Dryden Wind Gust Models27/1(Wg) -> Gain95/1, Gain112/1  "wGust"
  Nz pilot calculation25/1(Pilot g force (g)) -> Pilot G force Scope25/1, Nz Pilot (g)25/1
  Nz pilot calculation27/1(Pilot g force (g)) -> Pilot G force Scope27/1, Nz Pilot (g)27/1
  Gain95/1 -> Sum46/1
  Aircraft Dynamics Model28/1(Vertical Velocity w (ft/sec)) -> Gain102/1, Nz pilot calculation28/1(w)  "w"
  Aircraft Dynamics Model25/1(Vertical Velocity w (ft/sec)) -> Gain109/1, Nz pilot calculation25/1(w)  "w"
  Sum46/1 -> Aircraft Dynamics Model27/3(Rotary Gust qGust (rad/sec))
  Gain96/1 -> alpha (rad)27/1, Angle of Attack27/1, Controller27/2(alpha (rad))
  Aircraft Dynamics Model27/2(Pitch Rate q (rad/sec)) -> Nz pilot calculation27/2(q), Controller27/3(q (rad/sec))  "q"
  u27/1 -> Sum47/2
  Gain112/1 -> Aircraft Dynamics Model27/2(Vertical Gust wGust (ft/sec))
  Pilot27/1 -> Sum47/1
  Gain110/1 -> Sum44/1
  Sum47/1 -> Stick Input27/1, Controller27/1(Stick Input (in))
  Aircraft Dynamics Model27/1(Vertical Velocity w (ft/sec)) -> Gain96/1, Nz pilot calculation27/1(w)  "w"
  Sum45/1 -> Stick Input26/1, Controller26/1(Stick Input (in))
  Gain113/1 -> Sum46/2
  u29/1 -> Sum51/2
  Sum43/1 -> Stick Input25/1, Controller25/1(Stick Input (in))
  Sum53/1 -> Stick Input21/1, Controller21/1(Stick Input (in))
  Aircraft Dynamics Model20/1(Vertical Velocity w (ft/sec)) -> Gain115/1, Nz pilot calculation20/1(w)  "w"
  Nz pilot calculation22/1(Pilot g force (g)) -> Pilot G force Scope22/1, Nz Pilot (g)22/1
  Gain119/1 -> Sum54/2
  Sum55/1 -> Stick Input22/1, Controller22/1(Stick Input (in))
  Gain106/1 -> Sum42/1
  Gain116/1 -> Sum52/1
  Pilot22/1 -> Sum55/1
  Gain118/1 -> Aircraft Dynamics Model22/2(Vertical Gust wGust (ft/sec))
  Aircraft Dynamics Model22/1(Vertical Velocity w (ft/sec)) -> Gain83/1, Nz pilot calculation22/1(w)  "w"
  Aircraft Dynamics Model22/2(Pitch Rate q (rad/sec)) -> Nz pilot calculation22/2(q), Controller22/3(q (rad/sec))  "q"
  Gain83/1 -> alpha (rad)22/1, Angle of Attack22/1, Controller22/2(alpha (rad))
  Dryden Wind Gust Models22/2(Qg) -> Gain119/1  "qGust"
  u22/1 -> Sum55/2
  Gain91/1 -> alpha (rad)24/1, Angle of Attack24/1, Controller24/2(alpha (rad))
  Dryden Wind Gust Models24/2(Qg) -> Gain88/1  "qGust"
  Controller23/1(Elevator Command (deg)) -> Actuator Model23/1
  Gain86/1 -> Sum56/1
  Nz pilot calculation23/1(Pilot g force (g)) -> Pilot G force Scope23/1, Nz Pilot (g)23/1
  Sum59/1 -> Stick Input24/1, Controller24/1(Stick Input (in))
  Nz pilot calculation24/1(Pilot g force (g)) -> Pilot G force Scope24/1, Nz Pilot (g)24/1
  Actuator Model22/1 -> Aircraft Dynamics Model22/1(Elevator Deflection d (deg))
  Gain85/1 -> Sum56/2
  Aircraft Dynamics Model23/1(Vertical Velocity w (ft/sec)) -> Gain89/1, Nz pilot calculation23/1(w)  "w"
  Dryden Wind Gust Models27/2(Qg) -> Gain113/1  "qGust"
  Pilot24/1 -> Sum59/1
  Sum57/1 -> Stick Input23/1, Controller23/1(Stick Input (in))
  Aircraft Dynamics Model24/1(Vertical Velocity w (ft/sec)) -> Gain91/1, Nz pilot calculation24/1(w)  "w"
  Dryden Wind Gust Models23/1(Wg) -> Gain86/1, Gain84/1  "wGust"
  Aircraft Dynamics Model23/2(Pitch Rate q (rad/sec)) -> Nz pilot calculation23/2(q), Controller23/3(q (rad/sec))  "q"
  Dryden Wind Gust Models23/2(Qg) -> Gain85/1  "qGust"
  Actuator Model23/1 -> Aircraft Dynamics Model23/1(Elevator Deflection d (deg))
  Sum56/1 -> Aircraft Dynamics Model23/3(Rotary Gust qGust (rad/sec))
  Actuator Model24/1 -> Aircraft Dynamics Model24/1(Elevator Deflection d (deg))
  Gain84/1 -> Aircraft Dynamics Model23/2(Vertical Gust wGust (ft/sec))
  Gain89/1 -> alpha (rad)23/1, Angle of Attack23/1, Controller23/2(alpha (rad))
  Controller24/1(Elevator Command (deg)) -> Actuator Model24/1
  Gain90/1 -> Sum58/1
  Aircraft Dynamics Model24/2(Pitch Rate q (rad/sec)) -> Nz pilot calculation24/2(q), Controller24/3(q (rad/sec))  "q"
  Gain111/1 -> alpha (rad)26/1, Angle of Attack26/1, Controller26/2(alpha (rad))
  Gain87/1 -> Aircraft Dynamics Model24/2(Vertical Gust wGust (ft/sec))
  u24/1 -> Sum59/2
  u23/1 -> Sum57/2
  Controller27/1(Elevator Command (deg)) -> Actuator Model27/1
  Dryden Wind Gust Models24/1(Wg) -> Gain90/1, Gain87/1  "wGust"
  Aircraft Dynamics Model21/2(Pitch Rate q (rad/sec)) -> Nz pilot calculation21/2(q), Controller21/3(q (rad/sec))  "q"
  Sum58/1 -> Aircraft Dynamics Model24/3(Rotary Gust qGust (rad/sec))
  Gain97/1 -> Aircraft Dynamics Model28/2(Vertical Gust wGust (ft/sec))
  Gain93/1 -> Aircraft Dynamics Model25/2(Vertical Gust wGust (ft/sec))
  Pilot25/1 -> Sum43/1
  Gain94/1 -> Sum42/2
  u25/1 -> Sum43/2
  Nz pilot calculation26/1(Pilot g force (g)) -> Pilot G force Scope26/1, Nz Pilot (g)26/1
  Gain82/1 -> Sum54/1
  Dryden Wind Gust Models26/1(Wg) -> Gain110/1, Gain107/1  "wGust"
  Actuator Model26/1 -> Aircraft Dynamics Model26/1(Elevator Deflection d (deg))
  Gain117/1 -> alpha (rad)21/1, Angle of Attack21/1, Controller21/2(alpha (rad))
  Controller20/1(Elevator Command (deg)) -> Actuator Model20/1
  Gain108/1 -> Sum44/2
  Sum44/1 -> Aircraft Dynamics Model26/3(Rotary Gust qGust (rad/sec))
  Aircraft Dynamics Model26/1(Vertical Velocity w (ft/sec)) -> Gain111/1, Nz pilot calculation26/1(w)  "w"
  Dryden Wind Gust Models22/1(Wg) -> Gain82/1, Gain118/1  "wGust"
  Gain107/1 -> Aircraft Dynamics Model26/2(Vertical Gust wGust (ft/sec))
  Dryden Wind Gust Models20/1(Wg) -> Gain92/1, Gain80/1  "wGust"
  Gain109/1 -> alpha (rad)25/1, Angle of Attack25/1, Controller25/2(alpha (rad))
  Gain92/1 -> Sum40/1
  Aircraft Dynamics Model26/2(Pitch Rate q (rad/sec)) -> Nz pilot calculation26/2(q), Controller26/3(q (rad/sec))  "q"
  Nz pilot calculation20/1(Pilot g force (g)) -> Pilot G force Scope20/1, Nz Pilot (g)20/1
  Dryden Wind Gust Models28/2(Qg) -> Gain98/1  "qGust"
  Aircraft Dynamics Model25/2(Pitch Rate q (rad/sec)) -> Nz pilot calculation25/2(q), Controller25/3(q (rad/sec))  "q"
  Gain88/1 -> Sum58/2
  Pilot26/1 -> Sum45/1
  Dryden Wind Gust Models25/2(Qg) -> Gain94/1  "qGust"
  Actuator Model25/1 -> Aircraft Dynamics Model25/1(Elevator Deflection d (deg))
  Pilot23/1 -> Sum57/1
  Controller26/1(Elevator Command (deg)) -> Actuator Model26/1
  Sum42/1 -> Aircraft Dynamics Model25/3(Rotary Gust qGust (rad/sec))
  Gain105/1 -> alpha (rad)29/1, Angle of Attack29/1, Controller29/2(alpha (rad))
  Dryden Wind Gust Models26/2(Qg) -> Gain108/1  "qGust"
  Aircraft Dynamics Model21/1(Vertical Velocity w (ft/sec)) -> Gain117/1, Nz pilot calculation21/1(w)  "w"
  Controller29/1(Elevator Command (deg)) -> Actuator Model29/1
  Controller21/1(Elevator Command (deg)) -> Actuator Model21/1
  Pilot20/1 -> Sum41/1
  Sum51/1 -> Stick Input29/1, Controller29/1(Stick Input (in))
  u26/1 -> Sum45/2
  Sum49/1 -> Stick Input28/1, Controller28/1(Stick Input (in))
  Gain104/1 -> Sum50/1
  Nz pilot calculation29/1(Pilot g force (g)) -> Pilot G force Scope29/1, Nz Pilot (g)29/1
  Gain98/1 -> Sum48/2
  Pilot29/1 -> Sum51/1
  Actuator Model27/1 -> Aircraft Dynamics Model27/1(Elevator Deflection d (deg))
  Sum41/1 -> Stick Input20/1, Controller20/1(Stick Input (in))
  Gain100/1 -> Aircraft Dynamics Model29/2(Vertical Gust wGust (ft/sec))
  Controller22/1(Elevator Command (deg)) -> Actuator Model22/1
  Sum54/1 -> Aircraft Dynamics Model22/3(Rotary Gust qGust (rad/sec))
  Dryden Wind Gust Models29/2(Qg) -> Gain101/1  "qGust"
  Controller38/1(Elevator Command (deg)) -> Actuator Model38/1
  Gain143/1 -> Aircraft Dynamics Model31/2(Vertical Gust wGust (ft/sec))
  Dryden Wind Gust Models31/2(Qg) -> Gain154/1  "qGust"
  Actuator Model31/1 -> Aircraft Dynamics Model31/1(Elevator Deflection d (deg))
  Sum72/1 -> Aircraft Dynamics Model31/3(Rotary Gust qGust (rad/sec))
  Pilot31/1 -> Sum73/1
  Gain154/1 -> Sum72/2
  Nz pilot calculation31/1(Pilot g force (g)) -> Pilot G force Scope31/1, Nz Pilot (g)31/1
  Dryden Wind Gust Models31/1(Wg) -> Gain156/1, Gain143/1  "wGust"
  u30/1 -> Sum61/2
  Sum60/1 -> Aircraft Dynamics Model30/3(Rotary Gust qGust (rad/sec))
  Gain121/1 -> Sum60/2
  Gain155/1 -> alpha (rad)30/1, Angle of Attack30/1, Controller30/2(alpha (rad))
  Dryden Wind Gust Models30/2(Qg) -> Gain121/1  "qGust"
  Aircraft Dynamics Model30/2(Pitch Rate q (rad/sec)) -> Nz pilot calculation30/2(q), Controller30/3(q (rad/sec))  "q"
  Gain141/1 -> Sum70/2
  Dryden Wind Gust Models35/1(Wg) -> Gain146/1, Gain133/1  "wGust"
  Sum68/1 -> Aircraft Dynamics Model38/3(Rotary Gust qGust (rad/sec))
  u31/1 -> Sum73/2
  u38/1 -> Sum69/2
  Controller35/1(Elevator Command (deg)) -> Actuator Model35/1
  Actuator Model30/1 -> Aircraft Dynamics Model30/1(Elevator Deflection d (deg))
  Sum70/1 -> Aircraft Dynamics Model39/3(Rotary Gust qGust (rad/sec))
  Dryden Wind Gust Models39/1(Wg) -> Gain144/1, Gain140/1  "wGust"
  Aircraft Dynamics Model39/2(Pitch Rate q (rad/sec)) -> Nz pilot calculation39/2(q), Controller39/3(q (rad/sec))  "q"
  Gain142/1 -> alpha (rad)38/1, Angle of Attack38/1, Controller38/2(alpha (rad))
  Gain139/1 -> Sum68/1
  Nz pilot calculation38/1(Pilot g force (g)) -> Pilot G force Scope38/1, Nz Pilot (g)38/1
  Actuator Model38/1 -> Aircraft Dynamics Model38/1(Elevator Deflection d (deg))
  Dryden Wind Gust Models38/1(Wg) -> Gain139/1, Gain137/1  "wGust"
  Actuator Model39/1 -> Aircraft Dynamics Model39/1(Elevator Deflection d (deg))
  Pilot38/1 -> Sum69/1
  Aircraft Dynamics Model39/1(Vertical Velocity w (ft/sec)) -> Gain145/1, Nz pilot calculation39/1(w)  "w"
  Aircraft Dynamics Model38/2(Pitch Rate q (rad/sec)) -> Nz pilot calculation38/2(q), Controller38/3(q (rad/sec))  "q"
  Gain120/1 -> Aircraft Dynamics Model30/2(Vertical Gust wGust (ft/sec))
  Dryden Wind Gust Models37/1(Wg) -> Gain135/1, Gain152/1  "wGust"
  Nz pilot calculation35/1(Pilot g force (g)) -> Pilot G force Scope35/1, Nz Pilot (g)35/1
  Nz pilot calculation37/1(Pilot g force (g)) -> Pilot G force Scope37/1, Nz Pilot (g)37/1
  Gain135/1 -> Sum66/1
  Aircraft Dynamics Model38/1(Vertical Velocity w (ft/sec)) -> Gain142/1, Nz pilot calculation38/1(w)  "w"
  Aircraft Dynamics Model35/1(Vertical Velocity w (ft/sec)) -> Gain149/1, Nz pilot calculation35/1(w)  "w"
  Sum66/1 -> Aircraft Dynamics Model37/3(Rotary Gust qGust (rad/sec))
  Gain136/1 -> alpha (rad)37/1, Angle of Attack37/1, Controller37/2(alpha (rad))
  Aircraft Dynamics Model37/2(Pitch Rate q (rad/sec)) -> Nz pilot calculation37/2(q), Controller37/3(q (rad/sec))  "q"
  u37/1 -> Sum67/2
  Gain152/1 -> Aircraft Dynamics Model37/2(Vertical Gust wGust (ft/sec))
  Pilot37/1 -> Sum67/1
  Gain150/1 -> Sum64/1
  Sum67/1 -> Stick Input37/1, Controller37/1(Stick Input (in))
  Aircraft Dynamics Model37/1(Vertical Velocity w (ft/sec)) -> Gain136/1, Nz pilot calculation37/1(w)  "w"
  Sum65/1 -> Stick Input36/1, Controller36/1(Stick Input (in))
  Gain153/1 -> Sum66/2
  u39/1 -> Sum71/2
  Sum63/1 -> Stick Input35/1, Controller35/1(Stick Input (in))
  Sum73/1 -> Stick Input31/1, Controller31/1(Stick Input (in))
  Aircraft Dynamics Model30/1(Vertical Velocity w (ft/sec)) -> Gain155/1, Nz pilot calculation30/1(w)  "w"
  Nz pilot calculation32/1(Pilot g force (g)) -> Pilot G force Scope32/1, Nz Pilot (g)32/1
  Gain159/1 -> Sum74/2
  Sum75/1 -> Stick Input32/1, Controller32/1(Stick Input (in))
  Gain146/1 -> Sum62/1
  Gain156/1 -> Sum72/1
  Pilot32/1 -> Sum75/1
  Gain158/1 -> Aircraft Dynamics Model32/2(Vertical Gust wGust (ft/sec))
  Aircraft Dynamics Model32/1(Vertical Velocity w (ft/sec)) -> Gain123/1, Nz pilot calculation32/1(w)  "w"
  Aircraft Dynamics Model32/2(Pitch Rate q (rad/sec)) -> Nz pilot calculation32/2(q), Controller32/3(q (rad/sec))  "q"
  Gain123/1 -> alpha (rad)32/1, Angle of Attack32/1, Controller32/2(alpha (rad))
  Dryden Wind Gust Models32/2(Qg) -> Gain159/1  "qGust"
  u32/1 -> Sum75/2
  Gain131/1 -> alpha (rad)34/1, Angle of Attack34/1, Controller34/2(alpha (rad))
  Dryden Wind Gust Models34/2(Qg) -> Gain128/1  "qGust"
  Controller33/1(Elevator Command (deg)) -> Actuator Model33/1
  Gain126/1 -> Sum76/1
  Nz pilot calculation33/1(Pilot g force (g)) -> Pilot G force Scope33/1, Nz Pilot (g)33/1
  Sum79/1 -> Stick Input34/1, Controller34/1(Stick Input (in))
  Nz pilot calculation34/1(Pilot g force (g)) -> Pilot G force Scope34/1, Nz Pilot (g)34/1
  Actuator Model32/1 -> Aircraft Dynamics Model32/1(Elevator Deflection d (deg))
  Gain125/1 -> Sum76/2
  Aircraft Dynamics Model33/1(Vertical Velocity w (ft/sec)) -> Gain129/1, Nz pilot calculation33/1(w)  "w"
  Dryden Wind Gust Models37/2(Qg) -> Gain153/1  "qGust"
  Pilot34/1 -> Sum79/1
  Sum77/1 -> Stick Input33/1, Controller33/1(Stick Input (in))
  Aircraft Dynamics Model34/1(Vertical Velocity w (ft/sec)) -> Gain131/1, Nz pilot calculation34/1(w)  "w"
  Dryden Wind Gust Models33/1(Wg) -> Gain126/1, Gain124/1  "wGust"
  Aircraft Dynamics Model33/2(Pitch Rate q (rad/sec)) -> Nz pilot calculation33/2(q), Controller33/3(q (rad/sec))  "q"
  Dryden Wind Gust Models33/2(Qg) -> Gain125/1  "qGust"
  Actuator Model33/1 -> Aircraft Dynamics Model33/1(Elevator Deflection d (deg))
  Sum76/1 -> Aircraft Dynamics Model33/3(Rotary Gust qGust (rad/sec))
  Actuator Model34/1 -> Aircraft Dynamics Model34/1(Elevator Deflection d (deg))
  Gain124/1 -> Aircraft Dynamics Model33/2(Vertical Gust wGust (ft/sec))
  Gain129/1 -> alpha (rad)33/1, Angle of Attack33/1, Controller33/2(alpha (rad))
  Controller34/1(Elevator Command (deg)) -> Actuator Model34/1
  Gain130/1 -> Sum78/1
  Aircraft Dynamics Model34/2(Pitch Rate q (rad/sec)) -> Nz pilot calculation34/2(q), Controller34/3(q (rad/sec))  "q"
  Gain151/1 -> alpha (rad)36/1, Angle of Attack36/1, Controller36/2(alpha (rad))
  Gain127/1 -> Aircraft Dynamics Model34/2(Vertical Gust wGust (ft/sec))
  u34/1 -> Sum79/2
  u33/1 -> Sum77/2
  Controller37/1(Elevator Command (deg)) -> Actuator Model37/1
  Dryden Wind Gust Models34/1(Wg) -> Gain130/1, Gain127/1  "wGust"
  Aircraft Dynamics Model31/2(Pitch Rate q (rad/sec)) -> Nz pilot calculation31/2(q), Controller31/3(q (rad/sec))  "q"
  Sum78/1 -> Aircraft Dynamics Model34/3(Rotary Gust qGust (rad/sec))
  Gain137/1 -> Aircraft Dynamics Model38/2(Vertical Gust wGust (ft/sec))
  Gain133/1 -> Aircraft Dynamics Model35/2(Vertical Gust wGust (ft/sec))
  Pilot35/1 -> Sum63/1
  Gain134/1 -> Sum62/2
  u35/1 -> Sum63/2
  Nz pilot calculation36/1(Pilot g force (g)) -> Pilot G force Scope36/1, Nz Pilot (g)36/1
  Gain122/1 -> Sum74/1
  Dryden Wind Gust Models36/1(Wg) -> Gain150/1, Gain147/1  "wGust"
  Actuator Model36/1 -> Aircraft Dynamics Model36/1(Elevator Deflection d (deg))
  Gain157/1 -> alpha (rad)31/1, Angle of Attack31/1, Controller31/2(alpha (rad))
  Controller30/1(Elevator Command (deg)) -> Actuator Model30/1
  Gain148/1 -> Sum64/2
  Sum64/1 -> Aircraft Dynamics Model36/3(Rotary Gust qGust (rad/sec))
  Aircraft Dynamics Model36/1(Vertical Velocity w (ft/sec)) -> Gain151/1, Nz pilot calculation36/1(w)  "w"
  Dryden Wind Gust Models32/1(Wg) -> Gain122/1, Gain158/1  "wGust"
  Gain147/1 -> Aircraft Dynamics Model36/2(Vertical Gust wGust (ft/sec))
  Dryden Wind Gust Models30/1(Wg) -> Gain132/1, Gain120/1  "wGust"
  Gain149/1 -> alpha (rad)35/1, Angle of Attack35/1, Controller35/2(alpha (rad))
  Gain132/1 -> Sum60/1
  Aircraft Dynamics Model36/2(Pitch Rate q (rad/sec)) -> Nz pilot calculation36/2(q), Controller36/3(q (rad/sec))  "q"
  Nz pilot calculation30/1(Pilot g force (g)) -> Pilot G force Scope30/1, Nz Pilot (g)30/1
  Dryden Wind Gust Models38/2(Qg) -> Gain138/1  "qGust"
  Aircraft Dynamics Model35/2(Pitch Rate q (rad/sec)) -> Nz pilot calculation35/2(q), Controller35/3(q (rad/sec))  "q"
  Gain128/1 -> Sum78/2
  Pilot36/1 -> Sum65/1
  Dryden Wind Gust Models35/2(Qg) -> Gain134/1  "qGust"
  Actuator Model35/1 -> Aircraft Dynamics Model35/1(Elevator Deflection d (deg))
  Pilot33/1 -> Sum77/1
  Controller36/1(Elevator Command (deg)) -> Actuator Model36/1
  Sum62/1 -> Aircraft Dynamics Model35/3(Rotary Gust qGust (rad/sec))
  Gain145/1 -> alpha (rad)39/1, Angle of Attack39/1, Controller39/2(alpha (rad))
  Dryden Wind Gust Models36/2(Qg) -> Gain148/1  "qGust"
  Aircraft Dynamics Model31/1(Vertical Velocity w (ft/sec)) -> Gain157/1, Nz pilot calculation31/1(w)  "w"
  Controller39/1(Elevator Command (deg)) -> Actuator Model39/1
  Controller31/1(Elevator Command (deg)) -> Actuator Model31/1
  Pilot30/1 -> Sum61/1
  Sum71/1 -> Stick Input39/1, Controller39/1(Stick Input (in))
  u36/1 -> Sum65/2
  Sum69/1 -> Stick Input38/1, Controller38/1(Stick Input (in))
  Gain144/1 -> Sum70/1
  Nz pilot calculation39/1(Pilot g force (g)) -> Pilot G force Scope39/1, Nz Pilot (g)39/1
  Gain138/1 -> Sum68/2
  Pilot39/1 -> Sum71/1
  Actuator Model37/1 -> Aircraft Dynamics Model37/1(Elevator Deflection d (deg))
  Sum61/1 -> Stick Input30/1, Controller30/1(Stick Input (in))
  Gain140/1 -> Aircraft Dynamics Model39/2(Vertical Gust wGust (ft/sec))
  Controller32/1(Elevator Command (deg)) -> Actuator Model32/1
  Sum74/1 -> Aircraft Dynamics Model32/3(Rotary Gust qGust (rad/sec))
  Dryden Wind Gust Models39/2(Qg) -> Gain141/1  "qGust"
  Controller48/1(Elevator Command (deg)) -> Actuator Model48/1
  Gain183/1 -> Aircraft Dynamics Model41/2(Vertical Gust wGust (ft/sec))
  Dryden Wind Gust Models41/2(Qg) -> Gain194/1  "qGust"
  Actuator Model41/1 -> Aircraft Dynamics Model41/1(Elevator Deflection d (deg))
  Sum92/1 -> Aircraft Dynamics Model41/3(Rotary Gust qGust (rad/sec))
  Pilot41/1 -> Sum93/1
  Gain194/1 -> Sum92/2
  Nz pilot calculation41/1(Pilot g force (g)) -> Pilot G force Scope41/1, Nz Pilot (g)41/1
  Dryden Wind Gust Models41/1(Wg) -> Gain196/1, Gain183/1  "wGust"
  u40/1 -> Sum81/2
  Sum80/1 -> Aircraft Dynamics Model40/3(Rotary Gust qGust (rad/sec))
  Gain161/1 -> Sum80/2
  Gain195/1 -> alpha (rad)40/1, Angle of Attack40/1, Controller40/2(alpha (rad))
  Dryden Wind Gust Models40/2(Qg) -> Gain161/1  "qGust"
  Aircraft Dynamics Model40/2(Pitch Rate q (rad/sec)) -> Nz pilot calculation40/2(q), Controller40/3(q (rad/sec))  "q"
  Gain181/1 -> Sum90/2
  Dryden Wind Gust Models45/1(Wg) -> Gain186/1, Gain173/1  "wGust"
  Sum88/1 -> Aircraft Dynamics Model48/3(Rotary Gust qGust (rad/sec))
  u41/1 -> Sum93/2
  u48/1 -> Sum89/2
  Controller45/1(Elevator Command (deg)) -> Actuator Model45/1
  Actuator Model40/1 -> Aircraft Dynamics Model40/1(Elevator Deflection d (deg))
  Sum90/1 -> Aircraft Dynamics Model49/3(Rotary Gust qGust (rad/sec))
  Dryden Wind Gust Models49/1(Wg) -> Gain184/1, Gain180/1  "wGust"
  Aircraft Dynamics Model49/2(Pitch Rate q (rad/sec)) -> Nz pilot calculation49/2(q), Controller49/3(q (rad/sec))  "q"
  Gain182/1 -> alpha (rad)48/1, Angle of Attack48/1, Controller48/2(alpha (rad))
  Gain179/1 -> Sum88/1
  Nz pilot calculation48/1(Pilot g force (g)) -> Pilot G force Scope48/1, Nz Pilot (g)48/1
  Actuator Model48/1 -> Aircraft Dynamics Model48/1(Elevator Deflection d (deg))
  Dryden Wind Gust Models48/1(Wg) -> Gain179/1, Gain177/1  "wGust"
  Actuator Model49/1 -> Aircraft Dynamics Model49/1(Elevator Deflection d (deg))
  Pilot48/1 -> Sum89/1
  Aircraft Dynamics Model49/1(Vertical Velocity w (ft/sec)) -> Gain185/1, Nz pilot calculation49/1(w)  "w"
  Aircraft Dynamics Model48/2(Pitch Rate q (rad/sec)) -> Nz pilot calculation48/2(q), Controller48/3(q (rad/sec))  "q"
  Gain160/1 -> Aircraft Dynamics Model40/2(Vertical Gust wGust (ft/sec))
  Dryden Wind Gust Models47/1(Wg) -> Gain175/1, Gain192/1  "wGust"
  Nz pilot calculation45/1(Pilot g force (g)) -> Pilot G force Scope45/1, Nz Pilot (g)45/1
  Nz pilot calculation47/1(Pilot g force (g)) -> Pilot G force Scope47/1, Nz Pilot (g)47/1
  Gain175/1 -> Sum86/1
  Aircraft Dynamics Model48/1(Vertical Velocity w (ft/sec)) -> Gain182/1, Nz pilot calculation48/1(w)  "w"
  Aircraft Dynamics Model45/1(Vertical Velocity w (ft/sec)) -> Gain189/1, Nz pilot calculation45/1(w)  "w"
  Sum86/1 -> Aircraft Dynamics Model47/3(Rotary Gust qGust (rad/sec))
  Gain176/1 -> alpha (rad)47/1, Angle of Attack47/1, Controller47/2(alpha (rad))
  Aircraft Dynamics Model47/2(Pitch Rate q (rad/sec)) -> Nz pilot calculation47/2(q), Controller47/3(q (rad/sec))  "q"
  u47/1 -> Sum87/2
  Gain192/1 -> Aircraft Dynamics Model47/2(Vertical Gust wGust (ft/sec))
  Pilot47/1 -> Sum87/1
  Gain190/1 -> Sum84/1
  Sum87/1 -> Stick Input47/1, Controller47/1(Stick Input (in))
  Aircraft Dynamics Model47/1(Vertical Velocity w (ft/sec)) -> Gain176/1, Nz pilot calculation47/1(w)  "w"
  Sum85/1 -> Stick Input46/1, Controller46/1(Stick Input (in))
  Gain193/1 -> Sum86/2
  u49/1 -> Sum91/2
  Sum83/1 -> Stick Input45/1, Controller45/1(Stick Input (in))
  Sum93/1 -> Stick Input41/1, Controller41/1(Stick Input (in))
  Aircraft Dynamics Model40/1(Vertical Velocity w (ft/sec)) -> Gain195/1, Nz pilot calculation40/1(w)  "w"
  Nz pilot calculation42/1(Pilot g force (g)) -> Pilot G force Scope42/1, Nz Pilot (g)42/1
  Gain199/1 -> Sum94/2
  Sum95/1 -> Stick Input42/1, Controller42/1(Stick Input (in))
  Gain186/1 -> Sum82/1
  Gain196/1 -> Sum92/1
  Pilot42/1 -> Sum95/1
  Gain198/1 -> Aircraft Dynamics Model42/2(Vertical Gust wGust (ft/sec))
  Aircraft Dynamics Model42/1(Vertical Velocity w (ft/sec)) -> Gain163/1, Nz pilot calculation42/1(w)  "w"
  Aircraft Dynamics Model42/2(Pitch Rate q (rad/sec)) -> Nz pilot calculation42/2(q), Controller42/3(q (rad/sec))  "q"
  Gain163/1 -> alpha (rad)42/1, Angle of Attack42/1, Controller42/2(alpha (rad))
  Dryden Wind Gust Models42/2(Qg) -> Gain199/1  "qGust"
  u42/1 -> Sum95/2
  Gain171/1 -> alpha (rad)44/1, Angle of Attack44/1, Controller44/2(alpha (rad))
  Dryden Wind Gust Models44/2(Qg) -> Gain168/1  "qGust"
  Controller43/1(Elevator Command (deg)) -> Actuator Model43/1
  Gain166/1 -> Sum96/1
  Nz pilot calculation43/1(Pilot g force (g)) -> Pilot G force Scope43/1, Nz Pilot (g)43/1
  Sum99/1 -> Stick Input44/1, Controller44/1(Stick Input (in))
  Nz pilot calculation44/1(Pilot g force (g)) -> Pilot G force Scope44/1, Nz Pilot (g)44/1
  Actuator Model42/1 -> Aircraft Dynamics Model42/1(Elevator Deflection d (deg))
  Gain165/1 -> Sum96/2
  Aircraft Dynamics Model43/1(Vertical Velocity w (ft/sec)) -> Gain169/1, Nz pilot calculation43/1(w)  "w"
  Dryden Wind Gust Models47/2(Qg) -> Gain193/1  "qGust"
  Pilot44/1 -> Sum99/1
  Sum97/1 -> Stick Input43/1, Controller43/1(Stick Input (in))
  Aircraft Dynamics Model44/1(Vertical Velocity w (ft/sec)) -> Gain171/1, Nz pilot calculation44/1(w)  "w"
  Dryden Wind Gust Models43/1(Wg) -> Gain166/1, Gain164/1  "wGust"
  Aircraft Dynamics Model43/2(Pitch Rate q (rad/sec)) -> Nz pilot calculation43/2(q), Controller43/3(q (rad/sec))  "q"
  Dryden Wind Gust Models43/2(Qg) -> Gain165/1  "qGust"
  Actuator Model43/1 -> Aircraft Dynamics Model43/1(Elevator Deflection d (deg))
  Sum96/1 -> Aircraft Dynamics Model43/3(Rotary Gust qGust (rad/sec))
  Actuator Model44/1 -> Aircraft Dynamics Model44/1(Elevator Deflection d (deg))
  Gain164/1 -> Aircraft Dynamics Model43/2(Vertical Gust wGust (ft/sec))
  Gain169/1 -> alpha (rad)43/1, Angle of Attack43/1, Controller43/2(alpha (rad))
  Controller44/1(Elevator Command (deg)) -> Actuator Model44/1
  Gain170/1 -> Sum98/1
  Aircraft Dynamics Model44/2(Pitch Rate q (rad/sec)) -> Nz pilot calculation44/2(q), Controller44/3(q (rad/sec))  "q"
  Gain191/1 -> alpha (rad)46/1, Angle of Attack46/1, Controller46/2(alpha (rad))
  Gain167/1 -> Aircraft Dynamics Model44/2(Vertical Gust wGust (ft/sec))
  u44/1 -> Sum99/2
  u43/1 -> Sum97/2
  Controller47/1(Elevator Command (deg)) -> Actuator Model47/1
  Dryden Wind Gust Models44/1(Wg) -> Gain170/1, Gain167/1  "wGust"
  Aircraft Dynamics Model41/2(Pitch Rate q (rad/sec)) -> Nz pilot calculation41/2(q), Controller41/3(q (rad/sec))  "q"
  Sum98/1 -> Aircraft Dynamics Model44/3(Rotary Gust qGust (rad/sec))
  Gain177/1 -> Aircraft Dynamics Model48/2(Vertical Gust wGust (ft/sec))
  Gain173/1 -> Aircraft Dynamics Model45/2(Vertical Gust wGust (ft/sec))
  Pilot45/1 -> Sum83/1
  Gain174/1 -> Sum82/2
  u45/1 -> Sum83/2
  Nz pilot calculation46/1(Pilot g force (g)) -> Pilot G force Scope46/1, Nz Pilot (g)46/1
  Gain162/1 -> Sum94/1
  Dryden Wind Gust Models46/1(Wg) -> Gain190/1, Gain187/1  "wGust"
  Actuator Model46/1 -> Aircraft Dynamics Model46/1(Elevator Deflection d (deg))
  Gain197/1 -> alpha (rad)41/1, Angle of Attack41/1, Controller41/2(alpha (rad))
  Controller40/1(Elevator Command (deg)) -> Actuator Model40/1
  Gain188/1 -> Sum84/2
  Sum84/1 -> Aircraft Dynamics Model46/3(Rotary Gust qGust (rad/sec))
  Aircraft Dynamics Model46/1(Vertical Velocity w (ft/sec)) -> Gain191/1, Nz pilot calculation46/1(w)  "w"
  Dryden Wind Gust Models42/1(Wg) -> Gain162/1, Gain198/1  "wGust"
  Gain187/1 -> Aircraft Dynamics Model46/2(Vertical Gust wGust (ft/sec))
  Dryden Wind Gust Models40/1(Wg) -> Gain172/1, Gain160/1  "wGust"
  Gain189/1 -> alpha (rad)45/1, Angle of Attack45/1, Controller45/2(alpha (rad))
  Gain172/1 -> Sum80/1
  Aircraft Dynamics Model46/2(Pitch Rate q (rad/sec)) -> Nz pilot calculation46/2(q), Controller46/3(q (rad/sec))  "q"
  Nz pilot calculation40/1(Pilot g force (g)) -> Pilot G force Scope40/1, Nz Pilot (g)40/1
  Dryden Wind Gust Models48/2(Qg) -> Gain178/1  "qGust"
  Aircraft Dynamics Model45/2(Pitch Rate q (rad/sec)) -> Nz pilot calculation45/2(q), Controller45/3(q (rad/sec))  "q"
  Gain168/1 -> Sum98/2
  Pilot46/1 -> Sum85/1
  Dryden Wind Gust Models45/2(Qg) -> Gain174/1  "qGust"
  Actuator Model45/1 -> Aircraft Dynamics Model45/1(Elevator Deflection d (deg))
  Pilot43/1 -> Sum97/1
  Controller46/1(Elevator Command (deg)) -> Actuator Model46/1
  Sum82/1 -> Aircraft Dynamics Model45/3(Rotary Gust qGust (rad/sec))
  Gain185/1 -> alpha (rad)49/1, Angle of Attack49/1, Controller49/2(alpha (rad))
  Dryden Wind Gust Models46/2(Qg) -> Gain188/1  "qGust"
  Aircraft Dynamics Model41/1(Vertical Velocity w (ft/sec)) -> Gain197/1, Nz pilot calculation41/1(w)  "w"
  Controller49/1(Elevator Command (deg)) -> Actuator Model49/1
  Controller41/1(Elevator Command (deg)) -> Actuator Model41/1
  Pilot40/1 -> Sum81/1
  Sum91/1 -> Stick Input49/1, Controller49/1(Stick Input (in))
  u46/1 -> Sum85/2
  Sum89/1 -> Stick Input48/1, Controller48/1(Stick Input (in))
  Gain184/1 -> Sum90/1
  Nz pilot calculation49/1(Pilot g force (g)) -> Pilot G force Scope49/1, Nz Pilot (g)49/1
  Gain178/1 -> Sum88/2
  Pilot49/1 -> Sum91/1
  Actuator Model47/1 -> Aircraft Dynamics Model47/1(Elevator Deflection d (deg))
  Sum81/1 -> Stick Input40/1, Controller40/1(Stick Input (in))
  Gain180/1 -> Aircraft Dynamics Model49/2(Vertical Gust wGust (ft/sec))
  Controller42/1(Elevator Command (deg)) -> Actuator Model42/1
  Sum94/1 -> Aircraft Dynamics Model42/3(Rotary Gust qGust (rad/sec))
  Dryden Wind Gust Models49/2(Qg) -> Gain181/1  "qGust"
  Aircraft Dynamics Model59/1(Vertical Velocity w (ft/sec)) -> Gain352/1, Nz pilot calculation59/1(w)  "w"
  Pilot59/1 -> Sum120/1
  Gain368/1 -> Sum117/1
  Sum118/1 -> Stick Input58/1, Controller58/1(Stick Input (in))
  Actuator Model54/1 -> Aircraft Dynamics Model54/1(Elevator Deflection d (deg))
  Dryden Wind Gust Models56/2(Qg) -> Gain343/1  "qGust"
  Gain347/1 -> alpha (rad)64/1, Angle of Attack56/1, Controller56/2(alpha (rad))
  u62/1 -> Sum129/2
  Gain338/1 -> alpha (rad)62/1, Angle of Attack54/1, Controller54/2(alpha (rad))
  Aircraft Dynamics Model54/2(Pitch Rate q (rad/sec)) -> Nz pilot calculation54/2(q), Controller54/3(q (rad/sec))  "q"
  Gain376/1 -> Aircraft Dynamics Model54/2(Vertical Gust wGust (ft/sec))
  Aircraft Dynamics Model54/1(Vertical Velocity w (ft/sec)) -> Gain338/1, Nz pilot calculation54/1(w)  "w"
  Pilot54/1 -> Sum129/1
  Sum129/1 -> Stick Input54/1, Controller54/1(Stick Input (in))
  Gain377/1 -> Sum128/2
  Sum127/1 -> Stick Input53/1, Controller53/1(Stick Input (in))
  Aircraft Dynamics Model52/1(Vertical Velocity w (ft/sec)) -> Gain373/1, Nz pilot calculation52/1(w)  "w"
  Dryden Wind Gust Models86/2(Qg) -> Gain306/1  "qGust"
  Gain294/1 -> Aircraft Dynamics Model86/2(Vertical Gust wGust (ft/sec))
  Controller93/1(Elevator Command (deg)) -> Actuator Model93/1
  Gain371/1 -> Sum119/2
  Sum192/1 -> Aircraft Dynamics Model86/3(Rotary Gust qGust (rad/sec))
  Controller72/1(Elevator Command (deg)) -> Actuator Model72/1
  Gain208/1 -> alpha (rad)79/1, Angle of Attack72/1, Controller72/2(alpha (rad))
  Aircraft Dynamics Model64/1(Vertical Velocity w (ft/sec)) -> Gain221/1, Nz pilot calculation64/1(w)  "w"
  Sum137/1 -> Aircraft Dynamics Model68/3(Rotary Gust qGust (rad/sec))
  Dryden Wind Gust Models68/2(Qg) -> Gain394/1  "qGust"
  Actuator Model68/1 -> Aircraft Dynamics Model68/1(Elevator Deflection d (deg))
  Pilot69/1 -> Sum140/1
  Dryden Wind Gust Models65/1(Wg) -> Gain381/1, Gain222/1  "wGust"
  Gain392/1 -> Sum135/1
  Gain212/1 -> alpha (rad)75/1, Angle of Attack68/1, Controller68/2(alpha (rad))
  Aircraft Dynamics Model69/1(Vertical Velocity w (ft/sec)) -> Gain215/1, Nz pilot calculation69/1(w)  "w"
  Sum139/1 -> Aircraft Dynamics Model69/3(Rotary Gust qGust (rad/sec))
  Dryden Wind Gust Models69/1(Wg) -> Gain214/1, Gain210/1  "wGust"
  Actuator Model69/1 -> Aircraft Dynamics Model69/1(Elevator Deflection d (deg))
  Gain381/1 -> Sum150/1
  Nz pilot calculation69/1(Pilot g force (g)) -> Pilot G force Scope69/1, Nz Pilot (g)76/1
  Pilot68/1 -> Sum138/1
  Gain393/1 -> Aircraft Dynamics Model68/2(Vertical Gust wGust (ft/sec))
  Aircraft Dynamics Model64/2(Pitch Rate q (rad/sec)) -> Nz pilot calculation64/2(q), Controller64/3(q (rad/sec))  "q"
  Gain386/1 -> Aircraft Dynamics Model67/2(Vertical Gust wGust (ft/sec))
  u73/1 -> Sum153/2
  u74/1 -> Sum155/2
  Dryden Wind Gust Models67/1(Wg) -> Gain390/1, Gain386/1  "wGust"
  Gain215/1 -> alpha (rad)76/1, Angle of Attack69/1, Controller69/2(alpha (rad))
  Actuator Model67/1 -> Aircraft Dynamics Model67/1(Elevator Deflection d (deg))
  Aircraft Dynamics Model66/2(Pitch Rate q (rad/sec)) -> Nz pilot calculation66/2(q), Controller66/3(q (rad/sec))  "q"
  Dryden Wind Gust Models66/2(Qg) -> Gain384/1  "qGust"
  Sum152/1 -> Aircraft Dynamics Model66/3(Rotary Gust qGust (rad/sec))
  Gain383/1 -> Aircraft Dynamics Model66/2(Vertical Gust wGust (ft/sec))
  Actuator Model66/1 -> Aircraft Dynamics Model66/1(Elevator Deflection d (deg))
  Gain388/1 -> alpha (rad)73/1, Angle of Attack66/1, Controller66/2(alpha (rad))
  Aircraft Dynamics Model67/1(Vertical Velocity w (ft/sec)) -> Gain391/1, Nz pilot calculation67/1(w)  "w"
  Sum153/1 -> Stick Input66/1, Controller66/1(Stick Input (in))
  Pilot67/1 -> Sum155/1
  Dryden Wind Gust Models70/2(Qg) -> Gain217/1  "qGust"
  Actuator Model65/1 -> Aircraft Dynamics Model65/1(Elevator Deflection d (deg))
  Nz pilot calculation66/1(Pilot g force (g)) -> Pilot G force Scope66/1, Nz Pilot (g)73/1
  Gain391/1 -> alpha (rad)74/1, Angle of Attack67/1, Controller67/2(alpha (rad))
  Sum155/1 -> Stick Input67/1, Controller67/1(Stick Input (in))
  Gain382/1 -> alpha (rad)72/1, Angle of Attack65/1, Controller65/2(alpha (rad))
  u72/1 -> Sum151/2
  Dryden Wind Gust Models72/2(Qg) -> Gain204/1  "qGust"
  Aircraft Dynamics Model67/2(Pitch Rate q (rad/sec)) -> Nz pilot calculation67/2(q), Controller67/3(q (rad/sec))  "q"
  Controller65/1(Elevator Command (deg)) -> Actuator Model65/1
  Pilot72/1 -> Sum147/1
  Sum150/1 -> Aircraft Dynamics Model65/3(Rotary Gust qGust (rad/sec))
  Sum136/1 -> Stick Input63/1, Controller63/1(Stick Input (in))
  Actuator Model70/1 -> Aircraft Dynamics Model70/1(Elevator Deflection d (deg))
  Gain207/1 -> Sum146/1
  Nz pilot calculation72/1(Pilot g force (g)) -> Pilot G force Scope72/1, Nz Pilot (g)79/1
  Gain398/1 -> Sum143/2
  u76/1 -> Sum140/2
  Gain323/1 -> Aircraft Dynamics Model51/2(Vertical Gust wGust (ft/sec))
  Dryden Wind Gust Models63/1(Wg) -> Gain392/1, Gain379/1  "wGust"
  Dryden Wind Gust Models51/2(Qg) -> Gain334/1  "qGust"
  Aircraft Dynamics Model51/2(Pitch Rate q (rad/sec)) -> Nz pilot calculation51/2(q), Controller51/3(q (rad/sec))  "q"
  Gain387/1 -> Sum154/2
  Actuator Model51/1 -> Aircraft Dynamics Model51/1(Elevator Deflection d (deg))
  Aircraft Dynamics Model53/2(Pitch Rate q (rad/sec)) -> Nz pilot calculation53/2(q), Controller53/3(q (rad/sec))  "q"
  Sum112/1 -> Aircraft Dynamics Model51/3(Rotary Gust qGust (rad/sec))
  u51/1 -> Sum123/2
  Gain342/1 -> Aircraft Dynamics Model56/2(Vertical Gust wGust (ft/sec))
  u63/1 -> Sum131/2
  Dryden Wind Gust Models58/1(Wg) -> Gain368/1, Gain364/1  "wGust"
  Gain337/1 -> Sum128/1
  Gain350/1 -> Sum115/2
  Gain353/1 -> Aircraft Dynamics Model60/2(Vertical Gust wGust (ft/sec))
  Gain334/1 -> Sum112/2
  Dryden Wind Gust Models51/1(Wg) -> Gain356/1, Gain323/1  "wGust"
  Controller51/1(Elevator Command (deg)) -> Actuator Model51/1
  u50/1 -> Sum101/2
  Gain201/1 -> Sum100/2
  Gain345/1 -> alpha (rad)50/1, Angle of Attack50/1, Controller50/2(alpha (rad))
  Aircraft Dynamics Model50/2(Pitch Rate q (rad/sec)) -> Nz pilot calculation50/2(q), Controller50/3(q (rad/sec))  "q"
  Pilot50/1 -> Sum101/1
  Gain321/1 -> Sum110/2
  u59/1 -> Sum111/2
  Aircraft Dynamics Model96/2(Pitch Rate q (rad/sec)) -> Nz pilot calculation96/2(q), Controller96/3(q (rad/sec))  "q"
  Gain331/1 -> alpha (rad)56/1, Angle of Attack96/1, Controller96/2(alpha (rad))
  u58/1 -> Sum109/2
  Controller95/1(Elevator Command (deg)) -> Actuator Model95/1
  Sum110/1 -> Aircraft Dynamics Model99/3(Rotary Gust qGust (rad/sec))
  Dryden Wind Gust Models99/1(Wg) -> Gain324/1, Gain320/1  "wGust"
  Gain320/1 -> Aircraft Dynamics Model99/2(Vertical Gust wGust (ft/sec))
  Gain324/1 -> Sum110/1
  Nz pilot calculation63/1(Pilot g force (g)) -> Pilot G force Scope63/1, Nz Pilot (g)70/1
  Aircraft Dynamics Model99/2(Pitch Rate q (rad/sec)) -> Nz pilot calculation99/2(q), Controller99/3(q (rad/sec))  "q"
  Controller99/1(Elevator Command (deg)) -> Actuator Model99/1
  Gain322/1 -> alpha (rad)58/1, Angle of Attack98/1, Controller98/2(alpha (rad))
  Nz pilot calculation98/1(Pilot g force (g)) -> Pilot G force Scope98/1, Nz Pilot (g)58/1
  Gain370/1 -> Aircraft Dynamics Model59/2(Vertical Gust wGust (ft/sec))
  Actuator Model99/1 -> Aircraft Dynamics Model99/1(Elevator Deflection d (deg))
  Nz pilot calculation54/1(Pilot g force (g)) -> Pilot G force Scope54/1, Nz Pilot (g)62/1
  Dryden Wind Gust Models98/2(Qg) -> Gain318/1  "qGust"
  Aircraft Dynamics Model98/2(Pitch Rate q (rad/sec)) -> Nz pilot calculation98/2(q), Controller98/3(q (rad/sec))  "q"
  Gain200/1 -> Aircraft Dynamics Model50/2(Vertical Gust wGust (ft/sec))
  Nz pilot calculation97/1(Pilot g force (g)) -> Pilot G force Scope97/1, Nz Pilot (g)57/1
  Aircraft Dynamics Model95/1(Vertical Velocity w (ft/sec)) -> Gain329/1, Nz pilot calculation95/1(w)  "w"
  Gain316/1 -> alpha (rad)57/1, Angle of Attack97/1, Controller97/2(alpha (rad))
  Aircraft Dynamics Model97/2(Pitch Rate q (rad/sec)) -> Nz pilot calculation97/2(q), Controller97/3(q (rad/sec))  "q"
  Gain390/1 -> Sum154/1
  u57/1 -> Sum107/2
  Pilot97/1 -> Sum107/1
  Gain330/1 -> Sum104/1
  Sum107/1 -> Stick Input97/1, Controller97/1(Stick Input (in))
  Aircraft Dynamics Model97/1(Vertical Velocity w (ft/sec)) -> Gain316/1, Nz pilot calculation97/1(w)  "w"
  Sum105/1 -> Stick Input96/1, Controller96/1(Stick Input (in))
  Sum145/1 -> Stick Input62/1, Controller62/1(Stick Input (in))
  Gain326/1 -> Sum102/1
  Gain356/1 -> Sum112/1
  Aircraft Dynamics Model62/1(Vertical Velocity w (ft/sec)) -> Gain213/1, Nz pilot calculation62/1(w)  "w"
  Gain385/1 -> Sum152/1
  Gain325/1 -> alpha (rad)59/1, Angle of Attack99/1, Controller99/2(alpha (rad))
  Sum114/1 -> Stick Input52/1, Controller52/1(Stick Input (in))
  Nz pilot calculation67/1(Pilot g force (g)) -> Pilot G force Scope67/1, Nz Pilot (g)74/1
  Actuator Model59/1 -> Aircraft Dynamics Model59/1(Elevator Deflection d (deg))
  Gain357/1 -> Aircraft Dynamics Model61/2(Vertical Gust wGust (ft/sec))
  Sum125/1 -> Stick Input61/1, Controller61/1(Stick Input (in))
  Controller53/1(Elevator Command (deg)) -> Actuator Model53/1
  Pilot51/1 -> Sum123/1
  Sum122/1 -> Stick Input60/1, Controller60/1(Stick Input (in))
  Nz pilot calculation61/1(Pilot g force (g)) -> Pilot G force Scope61/1, Nz Pilot (g)69/1
  Gain317/1 -> Aircraft Dynamics Model98/2(Vertical Gust wGust (ft/sec))
  Aircraft Dynamics Model55/1(Vertical Velocity w (ft/sec)) -> Gain344/1, Nz pilot calculation55/1(w)  "w"
  Sum115/1 -> Aircraft Dynamics Model57/3(Rotary Gust qGust (rad/sec))
  Dryden Wind Gust Models58/2(Qg) -> Gain365/1  "qGust"
  Dryden Wind Gust Models57/2(Qg) -> Gain350/1  "qGust"
  Pilot58/1 -> Sum118/1
  Aircraft Dynamics Model57/2(Pitch Rate q (rad/sec)) -> Nz pilot calculation57/2(q), Controller57/3(q (rad/sec))  "q"
  Nz pilot calculation52/1(Pilot g force (g)) -> Pilot G force Scope52/1, Nz Pilot (g)60/1
  Dryden Wind Gust Models52/1(Wg) -> Gain348/1, Gain335/1  "wGust"
  Dryden Wind Gust Models84/2(Qg) -> Gain268/1  "qGust"
  Gain246/1 -> Sum156/1
  Nz pilot calculation73/1(Pilot g force (g)) -> Pilot G force Scope73/1, Nz Pilot (g)53/1
  Gain343/1 -> Sum132/2
  Gain235/1 -> Sum156/2
  Aircraft Dynamics Model73/2(Pitch Rate q (rad/sec)) -> Nz pilot calculation73/2(q), Controller73/3(q (rad/sec))  "q"
  u65/1 -> Sum116/2
  Actuator Model86/1 -> Aircraft Dynamics Model86/1(Elevator Deflection d (deg))
  Dryden Wind Gust Models73/2(Qg) -> Gain235/1  "qGust"
  Actuator Model73/1 -> Aircraft Dynamics Model73/1(Elevator Deflection d (deg))
  Gain224/1 -> Aircraft Dynamics Model73/2(Vertical Gust wGust (ft/sec))
  Gain290/1 -> Sum178/1
  Aircraft Dynamics Model84/2(Pitch Rate q (rad/sec)) -> Nz pilot calculation84/2(q), Controller84/3(q (rad/sec))  "q"
  u54/1 -> Sum189/2
  u53/1 -> Sum167/2
  Controller97/1(Elevator Command (deg)) -> Actuator Model97/1
  Nz pilot calculation87/1(Pilot g force (g)) -> Pilot G force Scope87/1, Nz Pilot (g)92/1
  Gain340/1 -> Sum130/2
  Sum195/1 -> Stick Input87/1, Controller87/1(Stick Input (in))
  Gain374/1 -> Sum126/1
  Sum184/1 -> Stick Input91/1, Controller91/1(Stick Input (in))
  Gain305/1 -> Sum185/2
  Aircraft Dynamics Model58/2(Pitch Rate q (rad/sec)) -> Nz pilot calculation58/2(q), Controller58/3(q (rad/sec))  "q"
  Dryden Wind Gust Models62/2(Qg) -> Gain389/1  "qGust"
  u99/1 -> Sum191/2
  Aircraft Dynamics Model85/1(Vertical Velocity w (ft/sec)) -> Gain307/1, Nz pilot calculation85/1(w)  "w"
  Dryden Wind Gust Models94/2(Qg) -> Gain292/1  "qGust"
  Controller87/1(Elevator Command (deg)) -> Actuator Model87/1
  Gain291/1 -> Aircraft Dynamics Model94/2(Vertical Gust wGust (ft/sec))
  Sum191/1 -> Stick Input94/1, Controller94/1(Stick Input (in))
  Gain288/1 -> Sum187/2
  Sum180/1 -> Stick Input85/1, Controller85/1(Stick Input (in))
  Controller58/1(Elevator Command (deg)) -> Actuator Model58/1
  Gain295/1 -> Sum190/1
  Controller86/1(Elevator Command (deg)) -> Actuator Model86/1
  Gain362/1 -> alpha (rad)69/1, Angle of Attack61/1, Controller61/2(alpha (rad))
  Gain296/1 -> alpha (rad)99/1, Angle of Attack94/1, Controller94/2(alpha (rad))
  Dryden Wind Gust Models91/2(Qg) -> Gain299/1  "qGust"
  Nz pilot calculation55/1(Pilot g force (g)) -> Pilot G force Scope55/1, Nz Pilot (g)63/1
  Controller91/1(Elevator Command (deg)) -> Actuator Model91/1
  Aircraft Dynamics Model91/2(Pitch Rate q (rad/sec)) -> Nz pilot calculation91/2(q), Controller91/3(q (rad/sec))  "q"
  Nz pilot calculation85/1(Pilot g force (g)) -> Pilot G force Scope85/1, Nz Pilot (g)90/1
  Actuator Model90/1 -> Aircraft Dynamics Model90/1(Elevator Deflection d (deg))
  Gain300/1 -> alpha (rad)95/1, Angle of Attack90/1, Controller90/2(alpha (rad))
  Dryden Wind Gust Models97/1(Wg) -> Gain315/1, Gain332/1  "wGust"
  Nz pilot calculation95/1(Pilot g force (g)) -> Pilot G force Scope95/1, Nz Pilot (g)55/1
  Gain298/1 -> Aircraft Dynamics Model91/2(Vertical Gust wGust (ft/sec))
  Gain282/1 -> Sum179/1
  Gain271/1 -> Sum194/1
  Sum108/1 -> Aircraft Dynamics Model98/3(Rotary Gust qGust (rad/sec))
  Sum183/1 -> Aircraft Dynamics Model91/3(Rotary Gust qGust (rad/sec))
  Controller54/1(Elevator Command (deg)) -> Actuator Model54/1
  Dryden Wind Gust Models91/1(Wg) -> Gain302/1, Gain298/1  "wGust"
  Aircraft Dynamics Model53/1(Vertical Velocity w (ft/sec)) -> Gain375/1, Nz pilot calculation53/1(w)  "w"
  Gain299/1 -> Sum183/2
  Controller85/1(Elevator Command (deg)) -> Actuator Model85/1
  Aircraft Dynamics Model86/2(Pitch Rate q (rad/sec)) -> Nz pilot calculation86/2(q), Controller86/3(q (rad/sec))  "q"
  Controller64/1(Elevator Command (deg)) -> Actuator Model64/1
  Gain283/1 -> Aircraft Dynamics Model90/2(Vertical Gust wGust (ft/sec))
  Gain280/1 -> Sum198/1
  Aircraft Dynamics Model89/2(Pitch Rate q (rad/sec)) -> Nz pilot calculation89/2(q), Controller89/3(q (rad/sec))  "q"
  Controller89/1(Elevator Command (deg)) -> Actuator Model89/1
  u94/1 -> Sum199/2
  Gain278/1 -> alpha (rad)93/1, Angle of Attack88/1, Controller88/2(alpha (rad))
  Gain369/1 -> alpha (rad)66/1, Angle of Attack58/1, Controller58/2(alpha (rad))
  Actuator Model50/1 -> Aircraft Dynamics Model50/1(Elevator Deflection d (deg))
  Aircraft Dynamics Model88/2(Pitch Rate q (rad/sec)) -> Nz pilot calculation88/2(q), Controller88/3(q (rad/sec))  "q"
  Gain389/1 -> Sum134/2
  Actuator Model89/1 -> Aircraft Dynamics Model89/1(Elevator Deflection d (deg))
  Aircraft Dynamics Model62/2(Pitch Rate q (rad/sec)) -> Nz pilot calculation62/2(q), Controller62/3(q (rad/sec))  "q"
  Gain274/1 -> Sum196/2
  Actuator Model87/1 -> Aircraft Dynamics Model87/1(Elevator Deflection d (deg))
  Gain378/1 -> Aircraft Dynamics Model62/2(Vertical Gust wGust (ft/sec))
  Aircraft Dynamics Model89/1(Vertical Velocity w (ft/sec)) -> Gain281/1, Nz pilot calculation89/1(w)  "w"
  Dryden Wind Gust Models93/2(Qg) -> Gain288/1  "qGust"
  Aircraft Dynamics Model92/1(Vertical Velocity w (ft/sec)) -> Gain286/1, Nz pilot calculation92/1(w)  "w"
  Gain301/1 -> alpha (rad)54/1, Angle of Attack84/1, Controller84/2(alpha (rad))
  Gain275/1 -> Sum196/1
  Gain281/1 -> alpha (rad)94/1, Angle of Attack89/1, Controller89/2(alpha (rad))
  Nz pilot calculation88/1(Pilot g force (g)) -> Pilot G force Scope88/1, Nz Pilot (g)93/1
  Controller88/1(Elevator Command (deg)) -> Actuator Model88/1
  Dryden Wind Gust Models87/2(Qg) -> Gain311/1  "qGust"
  Aircraft Dynamics Model87/1(Vertical Velocity w (ft/sec)) -> Gain272/1, Nz pilot calculation87/1(w)  "w"
  Pilot87/1 -> Sum195/1
  Gain352/1 -> alpha (rad)67/1, Angle of Attack59/1, Controller59/2(alpha (rad))
  Pilot73/1 -> Sum167/1
  Actuator Model95/1 -> Aircraft Dynamics Model95/1(Elevator Deflection d (deg))
  Gain329/1 -> alpha (rad)55/1, Angle of Attack95/1, Controller95/2(alpha (rad))
  Dryden Wind Gust Models95/2(Qg) -> Gain314/1  "qGust"
  Gain313/1 -> Aircraft Dynamics Model95/2(Vertical Gust wGust (ft/sec))
  Pilot95/1 -> Sum103/1
  Gain314/1 -> Sum102/2
  u55/1 -> Sum103/2
  Actuator Model96/1 -> Aircraft Dynamics Model96/1(Elevator Deflection d (deg))
  Aircraft Dynamics Model96/1(Vertical Velocity w (ft/sec)) -> Gain331/1, Nz pilot calculation96/1(w)  "w"
  Dryden Wind Gust Models50/1(Wg) -> Gain312/1, Gain200/1  "wGust"
  Gain312/1 -> Sum100/1
  Gain220/1 -> Sum148/1
  Gain222/1 -> Aircraft Dynamics Model65/2(Vertical Gust wGust (ft/sec))
  Actuator Model58/1 -> Aircraft Dynamics Model58/1(Elevator Deflection d (deg))
  Dryden Wind Gust Models54/1(Wg) -> Gain337/1, Gain376/1  "wGust"
  u92/1 -> Sum195/2
  Pilot55/1 -> Sum131/1
  Pilot65/1 -> Sum151/1
  Sum149/1 -> Stick Input64/1, Controller64/1(Stick Input (in))
  Gain223/1 -> Sum150/2
  Gain375/1 -> alpha (rad)61/1, Angle of Attack53/1, Controller53/2(alpha (rad))
  Sum140/1 -> Stick Input69/1, Controller69/1(Stick Input (in))
  Sum194/1 -> Aircraft Dynamics Model87/3(Rotary Gust qGust (rad/sec))
  u79/1 -> Sum147/2
  Sum142/1 -> Stick Input70/1, Controller70/1(Stick Input (in))
  Nz pilot calculation65/1(Pilot g force (g)) -> Pilot G force Scope65/1, Nz Pilot (g)72/1
  Gain217/1 -> Sum141/2
  Gain214/1 -> Sum139/1
  Gain396/1 -> alpha (rad)77/1, Angle of Attack70/1, Controller70/2(alpha (rad))
  Dryden Wind Gust Models60/2(Qg) -> Gain354/1  "qGust"
  Gain216/1 -> Aircraft Dynamics Model70/2(Vertical Gust wGust (ft/sec))
  Actuator Model92/1 -> Aircraft Dynamics Model92/1(Elevator Deflection d (deg))
  Gain277/1 -> Sum198/2
  Gain297/1 -> Sum181/1
  u77/1 -> Sum142/2
  u67/1 -> Sum120/2
  Aircraft Dynamics Model68/1(Vertical Velocity w (ft/sec)) -> Gain212/1, Nz pilot calculation68/1(w)  "w"
  Aircraft Dynamics Model71/1(Vertical Velocity w (ft/sec)) -> Gain205/1, Nz pilot calculation71/1(w)  "w"
  Nz pilot calculation70/1(Pilot g force (g)) -> Pilot G force Scope70/1, Nz Pilot (g)77/1
  Gain395/1 -> Sum141/1
  Controller66/1(Elevator Command (deg)) -> Actuator Model66/1
  Nz pilot calculation62/1(Pilot g force (g)) -> Pilot G force Scope62/1, Nz Pilot (g)52/1
  Sum133/1 -> Stick Input56/1, Controller56/1(Stick Input (in))
  Gain379/1 -> Aircraft Dynamics Model63/2(Vertical Gust wGust (ft/sec))
  Gain284/1 -> Sum181/2
  Gain310/1 -> Aircraft Dynamics Model87/2(Vertical Gust wGust (ft/sec))
  Sum181/1 -> Aircraft Dynamics Model90/3(Rotary Gust qGust (rad/sec))
  Pilot71/1 -> Sum144/1
  Nz pilot calculation71/1(Pilot g force (g)) -> Pilot G force Scope71/1, Nz Pilot (g)78/1
  Gain349/1 -> Aircraft Dynamics Model57/2(Vertical Gust wGust (ft/sec))
  Dryden Wind Gust Models62/1(Wg) -> Gain202/1, Gain378/1  "wGust"
  Dryden Wind Gust Models71/1(Wg) -> Gain399/1, Gain397/1  "wGust"
  Dryden Wind Gust Models89/1(Wg) -> Gain280/1, Gain276/1  "wGust"
  Aircraft Dynamics Model72/2(Pitch Rate q (rad/sec)) -> Nz pilot calculation72/2(q), Controller72/3(q (rad/sec))  "q"
  Dryden Wind Gust Models96/1(Wg) -> Gain330/1, Gain327/1  "wGust"
  Gain205/1 -> alpha (rad)78/1, Angle of Attack71/1, Controller71/2(alpha (rad))
  Sum146/1 -> Aircraft Dynamics Model72/3(Rotary Gust qGust (rad/sec))
  Controller94/1(Elevator Command (deg)) -> Actuator Model94/1
  Actuator Model63/1 -> Aircraft Dynamics Model63/1(Elevator Deflection d (deg))
  u78/1 -> Sum144/2
  Dryden Wind Gust Models54/2(Qg) -> Gain377/1  "qGust"
  Gain204/1 -> Sum146/2
  Controller68/1(Elevator Command (deg)) -> Actuator Model68/1
  Dryden Wind Gust Models68/1(Wg) -> Gain209/1, Gain393/1  "wGust"
  Gain257/1 -> Aircraft Dynamics Model84/2(Vertical Gust wGust (ft/sec))
  Nz pilot calculation96/1(Pilot g force (g)) -> Pilot G force Scope96/1, Nz Pilot (g)56/1
  Sum189/1 -> Stick Input84/1, Controller84/1(Stick Input (in))
  Dryden Wind Gust Models50/2(Qg) -> Gain201/1  "qGust"
  Dryden Wind Gust Models63/2(Qg) -> Gain380/1  "qGust"
  Sum197/1 -> Stick Input88/1, Controller88/1(Stick Input (in))
  Dryden Wind Gust Models69/2(Qg) -> Gain211/1  "qGust"
  Actuator Model98/1 -> Aircraft Dynamics Model98/1(Elevator Deflection d (deg))
  Nz pilot calculation64/1(Pilot g force (g)) -> Pilot G force Scope64/1, Nz Pilot (g)71/1
  Sum100/1 -> Aircraft Dynamics Model50/3(Rotary Gust qGust (rad/sec))
  Pilot64/1 -> Sum149/1
  Gain218/1 -> Sum148/2
  Controller69/1(Elevator Command (deg)) -> Actuator Model69/1
  Nz pilot calculation50/1(Pilot g force (g)) -> Pilot G force Scope50/1, Nz Pilot (g)50/1
  Sum148/1 -> Aircraft Dynamics Model64/3(Rotary Gust qGust (rad/sec))
  Controller61/1(Elevator Command (deg)) -> Actuator Model61/1
  Pilot63/1 -> Sum136/1
  Actuator Model64/1 -> Aircraft Dynamics Model64/1(Elevator Deflection d (deg))
  Controller84/1(Elevator Command (deg)) -> Actuator Model84/1
  Dryden Wind Gust Models64/2(Qg) -> Gain218/1  "qGust"
  Dryden Wind Gust Models56/1(Wg) -> Gain346/1, Gain342/1  "wGust"
  Gain206/1 -> Aircraft Dynamics Model64/2(Vertical Gust wGust (ft/sec))
  Controller71/1(Elevator Command (deg)) -> Actuator Model71/1
  Actuator Model52/1 -> Aircraft Dynamics Model52/1(Elevator Deflection d (deg))
  Gain394/1 -> Sum137/2
  Gain202/1 -> Sum134/1
  Aircraft Dynamics Model91/1(Vertical Velocity w (ft/sec)) -> Gain303/1, Nz pilot calculation91/1(w)  "w"
  Dryden Wind Gust Models61/1(Wg) -> Gain361/1, Gain357/1  "wGust"
  Sum124/1 -> Aircraft Dynamics Model61/3(Rotary Gust qGust (rad/sec))
  Aircraft Dynamics Model90/2(Pitch Rate q (rad/sec)) -> Nz pilot calculation90/2(q), Controller90/3(q (rad/sec))  "q"
  Dryden Wind Gust Models57/1(Wg) -> Gain363/1, Gain349/1  "wGust"
  Dryden Wind Gust Models95/1(Wg) -> Gain326/1, Gain313/1  "wGust"
  Nz pilot calculation94/1(Pilot g force (g)) -> Pilot G force Scope94/1, Nz Pilot (g)99/1
  Gain336/1 -> Sum113/2
  u60/1 -> Sum114/2
  Dryden Wind Gust Models71/2(Qg) -> Gain398/1  "qGust"
  Gain348/1 -> Sum113/1
  Aircraft Dynamics Model95/2(Pitch Rate q (rad/sec)) -> Nz pilot calculation95/2(q), Controller95/3(q (rad/sec))  "q"
  Dryden Wind Gust Models53/1(Wg) -> Gain374/1, Gain360/1  "wGust"
  u68/1 -> Sum122/2
  Controller96/1(Elevator Command (deg)) -> Actuator Model96/1
  Aircraft Dynamics Model63/1(Vertical Velocity w (ft/sec)) -> Gain219/1, Nz pilot calculation63/1(w)  "w"
  Dryden Wind Gust Models53/2(Qg) -> Gain372/1  "qGust"
  Dryden Wind Gust Models61/2(Qg) -> Gain358/1  "qGust"
  Pilot60/1 -> Sum122/1
  Aircraft Dynamics Model61/1(Vertical Velocity w (ft/sec)) -> Gain362/1, Nz pilot calculation61/1(w)  "w"
  Dryden Wind Gust Models72/1(Wg) -> Gain207/1, Gain203/1  "wGust"
  Sum193/1 -> Stick Input86/1, Controller86/1(Stick Input (in))
  Gain399/1 -> Sum143/1
  Actuator Model61/1 -> Aircraft Dynamics Model61/1(Elevator Deflection d (deg))
  Sum119/1 -> Aircraft Dynamics Model59/3(Rotary Gust qGust (rad/sec))
  Aircraft Dynamics Model65/1(Vertical Velocity w (ft/sec)) -> Gain382/1, Nz pilot calculation65/1(w)  "w"
  Sum178/1 -> Aircraft Dynamics Model84/3(Rotary Gust qGust (rad/sec))
  Nz pilot calculation60/1(Pilot g force (g)) -> Pilot G force Scope60/1, Nz Pilot (g)68/1
  Gain359/1 -> alpha (rad)68/1, Angle of Attack60/1, Controller60/2(alpha (rad))
  Aircraft Dynamics Model71/2(Pitch Rate q (rad/sec)) -> Nz pilot calculation71/2(q), Controller71/3(q (rad/sec))  "q"
  Controller57/1(Elevator Command (deg)) -> Actuator Model57/1
  Pilot94/1 -> Sum191/1
  Gain253/1 -> Sum159/1
  Sum116/1 -> Stick Input57/1, Controller57/1(Stick Input (in))
  Gain266/1 -> Aircraft Dynamics Model76/2(Vertical Gust wGust (ft/sec))
  Aircraft Dynamics Model68/2(Pitch Rate q (rad/sec)) -> Nz pilot calculation68/2(q), Controller68/3(q (rad/sec))  "q"
  u95/1 -> Sum182/2
  Gain267/1 -> Sum172/2
  Gain261/1 -> Sum163/2
  u96/1 -> Sum184/2
  Sum182/1 -> Stick Input90/1, Controller90/1(Stick Input (in))
  u89/1 -> Sum169/2
  Sum171/1 -> Stick Input75/1, Controller75/1(Stick Input (in))
  Aircraft Dynamics Model74/1(Vertical Velocity w (ft/sec)) -> Gain263/1, Nz pilot calculation74/1(w)  "w"
  Aircraft Dynamics Model69/2(Pitch Rate q (rad/sec)) -> Nz pilot calculation69/2(q), Controller69/3(q (rad/sec))  "q"
  Gain258/1 -> Sum161/1
  Gain211/1 -> Sum139/2
  Controller63/1(Elevator Command (deg)) -> Actuator Model63/1
  Gain260/1 -> Aircraft Dynamics Model81/2(Vertical Gust wGust (ft/sec))
  Sum103/1 -> Stick Input95/1, Controller95/1(Stick Input (in))
  Pilot66/1 -> Sum153/1
  Gain276/1 -> Aircraft Dynamics Model89/2(Vertical Gust wGust (ft/sec))
  u87/1 -> Sum164/2
  Pilot81/1 -> Sum164/1
  Gain242/1 -> alpha (rad)87/1, Angle of Attack81/1, Controller81/2(alpha (rad))
  Pilot84/1 -> Sum189/1
  Controller52/1(Elevator Command (deg)) -> Actuator Model52/1
  Gain272/1 -> alpha (rad)92/1, Angle of Attack87/1, Controller87/2(alpha (rad))
  Dryden Wind Gust Models81/1(Wg) -> Gain241/1, Gain260/1  "wGust"
  Pilot82/1 -> Sum166/1
  Aircraft Dynamics Model82/2(Pitch Rate q (rad/sec)) -> Nz pilot calculation82/2(q), Controller82/3(q (rad/sec))  "q"
  Gain225/1 -> Aircraft Dynamics Model74/2(Vertical Gust wGust (ft/sec))
  Sum106/1 -> Aircraft Dynamics Model97/3(Rotary Gust qGust (rad/sec))
  Nz pilot calculation79/1(Pilot g force (g)) -> Pilot G force Scope79/1, Nz Pilot (g)85/1
  Gain315/1 -> Sum106/1
  Sum163/1 -> Aircraft Dynamics Model81/3(Rotary Gust qGust (rad/sec))
  Nz pilot calculation82/1(Pilot g force (g)) -> Pilot G force Scope82/1, Nz Pilot (g)88/1
  u70/1 -> Sum136/2
  Dryden Wind Gust Models52/2(Qg) -> Gain336/1  "qGust"
  Dryden Wind Gust Models82/1(Wg) -> Gain245/1, Gain243/1  "wGust"
  Sum151/1 -> Stick Input65/1, Controller65/1(Stick Input (in))
  Dryden Wind Gust Models66/1(Wg) -> Gain385/1, Gain383/1  "wGust"
  Sum156/1 -> Aircraft Dynamics Model73/3(Rotary Gust qGust (rad/sec))
  Nz pilot calculation58/1(Pilot g force (g)) -> Pilot G force Scope58/1, Nz Pilot (g)66/1
  Sum121/1 -> Aircraft Dynamics Model60/3(Rotary Gust qGust (rad/sec))
  Gain303/1 -> alpha (rad)96/1, Angle of Attack91/1, Controller91/2(alpha (rad))
  Dryden Wind Gust Models79/1(Wg) -> Gain253/1, Gain239/1  "wGust"
  Sum141/1 -> Aircraft Dynamics Model70/3(Rotary Gust qGust (rad/sec))
  u88/1 -> Sum166/2
  Sum165/1 -> Aircraft Dynamics Model82/3(Rotary Gust qGust (rad/sec))
  Gain341/1 -> Sum130/1
  Gain372/1 -> Sum126/2
  Actuator Model74/1 -> Aircraft Dynamics Model74/1(Elevator Deflection d (deg))
  Pilot61/1 -> Sum125/1
  u81/1 -> Sum171/2
  u75/1 -> Sum138/2
  Nz pilot calculation91/1(Pilot g force (g)) -> Pilot G force Scope91/1, Nz Pilot (g)96/1
  Actuator Model84/1 -> Aircraft Dynamics Model84/1(Elevator Deflection d (deg))
  Dryden Wind Gust Models73/1(Wg) -> Gain246/1, Gain224/1  "wGust"
  Gain226/1 -> Sum157/2
  Aircraft Dynamics Model79/1(Vertical Velocity w (ft/sec)) -> Gain256/1, Nz pilot calculation79/1(w)  "w"
  Dryden Wind Gust Models75/1(Wg) -> Gain264/1, Gain250/1  "wGust"
  Aircraft Dynamics Model74/2(Pitch Rate q (rad/sec)) -> Nz pilot calculation74/2(q), Controller74/3(q (rad/sec))  "q"
  Gain366/1 -> alpha (rad)65/1, Angle of Attack57/1, Controller57/2(alpha (rad))
  Pilot75/1 -> Sum171/1
  Aircraft Dynamics Model76/2(Pitch Rate q (rad/sec)) -> Nz pilot calculation76/2(q), Controller76/3(q (rad/sec))  "q"
  Nz pilot calculation75/1(Pilot g force (g)) -> Pilot G force Scope75/1, Nz Pilot (g)81/1
  Actuator Model57/1 -> Aircraft Dynamics Model57/1(Elevator Deflection d (deg))
  Gain332/1 -> Aircraft Dynamics Model97/2(Vertical Gust wGust (ft/sec))
  Gain251/1 -> Sum168/1
  Gain244/1 -> Sum165/2
  Sum198/1 -> Aircraft Dynamics Model89/3(Rotary Gust qGust (rad/sec))
  Nz pilot calculation83/1(Pilot g force (g)) -> Pilot G force Scope83/1, Nz Pilot (g)89/1
  Sum172/1 -> Aircraft Dynamics Model76/3(Rotary Gust qGust (rad/sec))
  u71/1 -> Sum149/2
  Pilot83/1 -> Sum169/1
  Dryden Wind Gust Models65/2(Qg) -> Gain223/1  "qGust"
  Gain247/1 -> Aircraft Dynamics Model83/2(Vertical Gust wGust (ft/sec))
  Sum158/1 -> Stick Input74/1, Controller74/1(Stick Input (in))
  Gain263/1 -> alpha (rad)80/1, Angle of Attack74/1, Controller74/2(alpha (rad))
  Pilot90/1 -> Sum182/1
  Gain268/1 -> Sum178/2
  Controller76/1(Elevator Command (deg)) -> Actuator Model76/1
  Pilot53/1 -> Sum127/1
  Pilot96/1 -> Sum105/1
  Sum170/1 -> Aircraft Dynamics Model75/3(Rotary Gust qGust (rad/sec))
  Dryden Wind Gust Models80/2(Qg) -> Gain255/1  "qGust"
  Controller75/1(Elevator Command (deg)) -> Actuator Model75/1
  Sum169/1 -> Stick Input83/1, Controller83/1(Stick Input (in))
  Dryden Wind Gust Models90/2(Qg) -> Gain284/1  "qGust"
  Pilot74/1 -> Sum158/1
  Aircraft Dynamics Model66/1(Vertical Velocity w (ft/sec)) -> Gain388/1, Nz pilot calculation66/1(w)  "w"
  u86/1 -> Sum162/2
  Controller83/1(Elevator Command (deg)) -> Actuator Model83/1
  Dryden Wind Gust Models83/2(Qg) -> Gain248/1  "qGust"
  Dryden Wind Gust Models59/2(Qg) -> Gain371/1  "qGust"
  Aircraft Dynamics Model60/1(Vertical Velocity w (ft/sec)) -> Gain359/1, Nz pilot calculation60/1(w)  "w"
  Gain252/1 -> alpha (rad)89/1, Angle of Attack83/1, Controller83/2(alpha (rad))
  Gain241/1 -> Sum163/1
  Sum159/1 -> Aircraft Dynamics Model79/3(Rotary Gust qGust (rad/sec))
  Gain210/1 -> Aircraft Dynamics Model69/2(Vertical Gust wGust (ft/sec))
  Actuator Model79/1 -> Aircraft Dynamics Model79/1(Elevator Deflection d (deg))
  Gain209/1 -> Sum137/1
  Pilot77/1 -> Sum175/1
  Aircraft Dynamics Model87/2(Pitch Rate q (rad/sec)) -> Nz pilot calculation87/2(q), Controller87/3(q (rad/sec))  "q"
  Aircraft Dynamics Model70/1(Vertical Velocity w (ft/sec)) -> Gain396/1, Nz pilot calculation70/1(w)  "w"
  Gain233/1 -> Sum176/2
  Aircraft Dynamics Model83/2(Pitch Rate q (rad/sec)) -> Nz pilot calculation83/2(q), Controller83/3(q (rad/sec))  "q"
  Nz pilot calculation74/1(Pilot g force (g)) -> Pilot G force Scope74/1, Nz Pilot (g)80/1
  Gain384/1 -> Sum152/2
  Aircraft Dynamics Model60/2(Pitch Rate q (rad/sec)) -> Nz pilot calculation60/2(q), Controller60/3(q (rad/sec))  "q"
  Gain238/1 -> Sum157/1
  Actuator Model53/1 -> Aircraft Dynamics Model53/1(Elevator Deflection d (deg))
  Aircraft Dynamics Model88/1(Vertical Velocity w (ft/sec)) -> Gain278/1, Nz pilot calculation88/1(w)  "w"
  Aircraft Dynamics Model70/2(Pitch Rate q (rad/sec)) -> Nz pilot calculation70/2(q), Controller70/3(q (rad/sec))  "q"
  u93/1 -> Sum197/2
  Controller74/1(Elevator Command (deg)) -> Actuator Model74/1
  Sum168/1 -> Aircraft Dynamics Model83/3(Rotary Gust qGust (rad/sec))
  Aircraft Dynamics Model99/1(Vertical Velocity w (ft/sec)) -> Gain325/1, Nz pilot calculation99/1(w)  "w"
  Gain265/1 -> alpha (rad)81/1, Angle of Attack75/1, Controller75/2(alpha (rad))
  Aircraft Dynamics Model50/1(Vertical Velocity w (ft/sec)) -> Gain345/1, Nz pilot calculation50/1(w)  "w"
  Aircraft Dynamics Model81/2(Pitch Rate q (rad/sec)) -> Nz pilot calculation81/2(q), Controller81/3(q (rad/sec))  "q"
  Gain254/1 -> Aircraft Dynamics Model80/2(Vertical Gust wGust (ft/sec))
  Pilot98/1 -> Sum109/1
  Gain363/1 -> Sum115/1
  Dryden Wind Gust Models74/2(Qg) -> Gain226/1  "qGust"
  Dryden Wind Gust Models76/1(Wg) -> Gain227/1, Gain266/1  "wGust"
  Gain311/1 -> Sum194/2
  Aircraft Dynamics Model80/1(Vertical Velocity w (ft/sec)) -> Gain259/1, Nz pilot calculation80/1(w)  "w"
  Sum161/1 -> Aircraft Dynamics Model80/3(Rotary Gust qGust (rad/sec))
  Gain255/1 -> Sum161/2
  Aircraft Dynamics Model65/2(Pitch Rate q (rad/sec)) -> Nz pilot calculation65/2(q), Controller65/3(q (rad/sec))  "q"
  Pilot85/1 -> Sum180/1
  Gain354/1 -> Sum121/2
  Controller59/1(Elevator Command (deg)) -> Actuator Model59/1
  Pilot79/1 -> Sum160/1
  Nz pilot calculation84/1(Pilot g force (g)) -> Pilot G force Scope84/1, Nz Pilot (g)54/1
  Actuator Model62/1 -> Aircraft Dynamics Model62/1(Elevator Deflection d (deg))
  Nz pilot calculation53/1(Pilot g force (g)) -> Pilot G force Scope53/1, Nz Pilot (g)61/1
  Gain227/1 -> Sum172/1
  Sum143/1 -> Aircraft Dynamics Model71/3(Rotary Gust qGust (rad/sec))
  Gain240/1 -> Sum159/2
  Dryden Wind Gust Models85/1(Wg) -> Gain282/1, Gain269/1  "wGust"
  Nz pilot calculation81/1(Pilot g force (g)) -> Pilot G force Scope81/1, Nz Pilot (g)87/1
  u85/1 -> Sum160/2
  Actuator Model80/1 -> Aircraft Dynamics Model80/1(Elevator Deflection d (deg))
  Gain239/1 -> Aircraft Dynamics Model79/2(Vertical Gust wGust (ft/sec))
  Gain264/1 -> Sum170/1
  Dryden Wind Gust Models78/1(Wg) -> Gain236/1, Gain232/1  "wGust"
  Pilot89/1 -> Sum199/1
  Pilot57/1 -> Sum116/1
  Aircraft Dynamics Model84/1(Vertical Velocity w (ft/sec)) -> Gain301/1, Nz pilot calculation84/1(w)  "w"
  Aircraft Dynamics Model81/1(Vertical Velocity w (ft/sec)) -> Gain242/1, Nz pilot calculation81/1(w)  "w"
  u83/1 -> Sum175/2
  Sum188/1 -> Stick Input93/1, Controller93/1(Stick Input (in))
  Sum160/1 -> Stick Input79/1, Controller79/1(Stick Input (in))
  u84/1 -> Sum177/2
  Gain243/1 -> Aircraft Dynamics Model82/2(Vertical Gust wGust (ft/sec))
  Gain232/1 -> Aircraft Dynamics Model78/2(Vertical Gust wGust (ft/sec))
  Controller81/1(Elevator Command (deg)) -> Actuator Model81/1
  u66/1 -> Sum118/2
  Controller50/1(Elevator Command (deg)) -> Actuator Model50/1
  Sum176/1 -> Aircraft Dynamics Model78/3(Rotary Gust qGust (rad/sec))
  Aircraft Dynamics Model78/2(Pitch Rate q (rad/sec)) -> Nz pilot calculation78/2(q), Controller78/3(q (rad/sec))  "q"
  Actuator Model82/1 -> Aircraft Dynamics Model82/1(Elevator Deflection d (deg))
  Pilot76/1 -> Sum173/1
  Actuator Model88/1 -> Aircraft Dynamics Model88/1(Elevator Deflection d (deg))
  Gain236/1 -> Sum176/1
  Controller60/1(Elevator Command (deg)) -> Actuator Model60/1
  Gain229/1 -> Aircraft Dynamics Model77/2(Vertical Gust wGust (ft/sec))
  Gain319/1 -> Sum108/1
  Controller78/1(Elevator Command (deg)) -> Actuator Model78/1
  Dryden Wind Gust Models75/2(Qg) -> Gain262/1  "qGust"
  Sum134/1 -> Aircraft Dynamics Model62/3(Rotary Gust qGust (rad/sec))
  Actuator Model77/1 -> Aircraft Dynamics Model77/1(Elevator Deflection d (deg))
  Gain203/1 -> Aircraft Dynamics Model72/2(Vertical Gust wGust (ft/sec))
  Sum174/1 -> Aircraft Dynamics Model77/3(Rotary Gust qGust (rad/sec))
  Actuator Model78/1 -> Aircraft Dynamics Model78/1(Elevator Deflection d (deg))
  Gain397/1 -> Aircraft Dynamics Model71/2(Vertical Gust wGust (ft/sec))
  Gain262/1 -> Sum170/2
  Aircraft Dynamics Model77/2(Pitch Rate q (rad/sec)) -> Nz pilot calculation77/2(q), Controller77/3(q (rad/sec))  "q"
  Gain328/1 -> Sum104/2
  Dryden Wind Gust Models77/2(Qg) -> Gain230/1  "qGust"
  Sum175/1 -> Stick Input77/1, Controller77/1(Stick Input (in))
  Aircraft Dynamics Model78/1(Vertical Velocity w (ft/sec)) -> Gain237/1, Nz pilot calculation78/1(w)  "w"
  Gain361/1 -> Sum124/1
  Gain273/1 -> Aircraft Dynamics Model88/2(Vertical Gust wGust (ft/sec))
  Dryden Wind Gust Models70/1(Wg) -> Gain395/1, Gain216/1  "wGust"
  Pilot78/1 -> Sum177/1
  Actuator Model83/1 -> Aircraft Dynamics Model83/1(Elevator Deflection d (deg))
  Dryden Wind Gust Models81/2(Qg) -> Gain261/1  "qGust"
  Gain230/1 -> Sum174/2
  Aircraft Dynamics Model80/2(Pitch Rate q (rad/sec)) -> Nz pilot calculation80/2(q), Controller80/3(q (rad/sec))  "q"
  Aircraft Dynamics Model83/1(Vertical Velocity w (ft/sec)) -> Gain252/1, Nz pilot calculation83/1(w)  "w"
  Aircraft Dynamics Model86/1(Vertical Velocity w (ft/sec)) -> Gain309/1, Nz pilot calculation86/1(w)  "w"
  Actuator Model76/1 -> Aircraft Dynamics Model76/1(Elevator Deflection d (deg))
  Aircraft Dynamics Model77/1(Vertical Velocity w (ft/sec)) -> Gain234/1, Nz pilot calculation77/1(w)  "w"
  Sum173/1 -> Stick Input76/1, Controller76/1(Stick Input (in))
